simulink model "Main"  (R2020b)
settings: Solver=FixedStepAuto  StartTime=0.0  StopTime=10  FixedStep=0.01  RelTol=1e-3
libraries: TcSimInterface x1
(part 1 of 2)
settings Model: Creator=kaebi  LastModifiedBy=kaebi
settings OptimizationCC: DefaultParameterBehavior=Inlined  LocalBlockOutputs=off
settings RTWCC: Description=TwinCAT GRT Target  SystemTargetFile=TwinCatGrt.tlc  GenCodeOnly=on  TemplateMakefile=tcgrt_msbuild.tmf  TargetLang=C++
settings STFCustomTargetCC: TargetLangStandard=C++03 (ISO)  ConcurrentExecutionCompliant=off  CombineOutputUpdateFcns=on  CodeInterfacePackaging=Reusable function  GRTInterface=off  GenerateAllocFcn=on  SystemTargetFile=TwinCatGrt.tlc
settings GRTTargetCC: TargetLangStandard=C++03 (ISO)  ParMdlRefBuildCompliant=off  CompOptLevelCompliant=off  ConcurrentExecutionCompliant=off  MatFileLogging=off  CodeInterfacePackaging=Reusable function  GenerateAllocFcn=on  UseToolchainInfoCompliant=off  ExtModeMexFile=TcExtModeClient

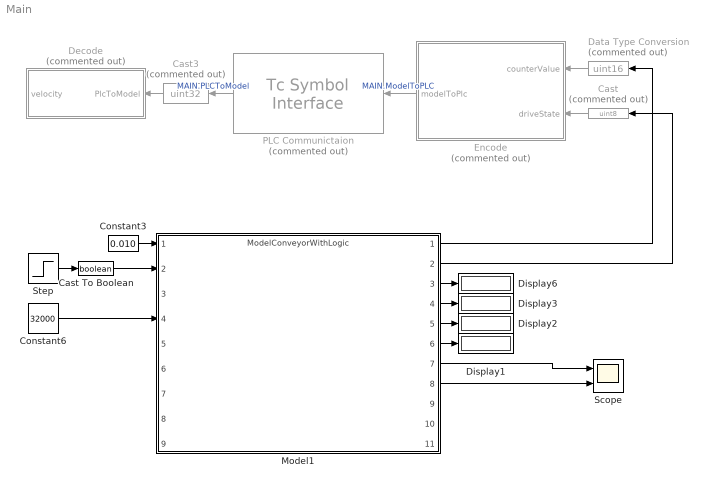
== system Main ==
  Cast : DataTypeConversion  Commented=on  OutDataTypeStr=uint8
  Cast To Boolean : DataTypeConversion  OutDataTypeStr=boolean
  Cast3 : DataTypeConversion  Commented=on  OutDataTypeStr=uint32
  Constant3 : Constant  Value=0.010
  Constant6 : Constant  Value=32000  OutDataTypeStr=int16
  Data Type Conversion : DataTypeConversion  Commented=on  OutDataTypeStr=uint16  SaturateOnIntegerOverflow=on
  Decode : MATLAB Function  Commented=on  TreatAsAtomicUnit=on
  Display{1..3,6} (4 alike) : Display
  Encode : MATLAB Function  Commented=on  TreatAsAtomicUnit=on
  Model1 : ModelReference  ModelNameDialog=ModelConveyorWithLogic.slx  SimulationMode=Normal  ModelReferenceVersion=1.29
  PLC Communictaion : TcSimInterface/Tc Symbol Interface  Commented=on  ChangeRowColOrder=on  TraceMode=3  DirectFeedThrough=0  SignalLabels=3  PortLabels=2  ExpandBusObjDepth=on  RuntimeConfig=|  SymbolInterfaceInfo=|  SyncClockMode=1
      RuntimeConfig=|
      | <?xml version="1.0" encoding="UTF-8" standalone="no"?>
      | <TcRuntimAdapterProject>
      | 	<DataTypes>
      | 		<DataType>
      | 			<Name GUID="{9165C8A1-78D1-4B81-89D0-BA48F61AF93B}" Namespace="TcDataExchange">ITcStreamSynchronizer</Name>
      | 			<Comment TxtId=""><![CDATA[Provides time synchronisation between data sources and data sinks in different time contexts. A time context might be a real time TwinCAT system the simulation time of a simulation tool or the basic time stamp of logged data in a database.]]></Comment>
      | 			<BitSize X64="64">32</BitSize>
      | 			<BaseType GUID="{00000001-0000-0000-E000-000000000064}">ITcUnknown</BaseType>
      | 			<Method>
      | 				<Name>RegisterTimeContext</Name>
      | 				<Comment><![CDATA[Registers a time context for synchronization. Registration has to be completet for all time contexts before starting the communication. ]]></Comment>
      | 				<ReturnType GUID="{18071995-0000-0000-0000-000000000019}">HRESULT</ReturnType>
      | 				<ReturnBitSize>32</ReturnBitSize>
      | 				<Parameter>
      | 					<Name>pSyncId</Name>
      | 					<Comment><![CDATA[Unique identifier of the time context. This might be e.g. the AmsNetId of a TwinCAT system or a ULINT representation of a logged dataset.]]></Comment>
      | 					<Type GUID="{18071995-0000-0000-0000-000000000021}" PointerTo="1">GUID</Type>
      | 					<BitSize X64="64">32</BitSize>
      | 				</Parameter>
      | 				<Parameter>
      | 					<Name>timeStamp</Name>
      | 					<Comment><![CDATA[Timestamp of the first received sample]]></Comment>
      | 					<Type GUID="{18071995-0000-0000-0000-00000000000C}">LINT</Type>
      | 					<BitSize>64</BitSize>
      | 				</Parameter>
      | 			</Method>
      | 			<Method>
      | 				<Name>TransformTime</Name>
      | 				<ReturnType GUID="{18071995-0000-0000-0000-000000000019}">HRESULT</ReturnType>
      | 				<ReturnBitSize>32</ReturnBitSize>
      | 				<Parameter>
      | 					<Name>pSourceSyncId</Name>
      | 					<Comment><![CDATA[Unique identifier of the source time context.]]></Comment>
      | 					<Type GUID="{18071995-0000-0000-0000-000000000021}" PointerTo="1">GUID</Type>
      | 					<BitSize X64="64">32</BitSize>
      | 				</Parameter>
      | 				<Parameter>
      | 					<Name>pSinkSyncId</Name>
      | 					<Comment><![CDATA[Unique identifier of the sink time context.]]></Comment>
      | 					<Type GUID="{18071995-0000-0000-0000-000000000021}" PointerTo="1">GUID</Type>
      | 					<BitSize X64="64">32</BitSize>
      | 				</Parameter>
      | 				<Parameter>
      | 					<Name>timeStamp</Name>
      | 					<Comment><![CDATA[Expects the sink timestamp and returns the appropriate source timestamp.
      | If the specified sink sync ID is unknown, the sink timestamp is register as its start time.]]></Comment>
      | 					<Type GUID="{18071995-0000-0000-0000-00000000000C}" ReferenceTo="true">LINT</Type>
      | 					<BitSize X64="64">32</BitSize>
      | 				</Parameter>
      | 			</Method>
      | 			<Hides>
      | 				<Hide GUID="{92EEAEA2-3DA4-48E7-A741-8C78A0326B08}"/>
      | 				<Hide GUID="{4F229E80-CBB0-4042-863E-770932FFF733}"/>
      | 				<Hide GUID="{BDB7FF6F-6144-4421-92B4-18BEEF6031E5}"/>
      | 				<Hide GUID="{5983EBFA-553B-4573-BA8B-8294D34A7664}"/>
      | 				<Hide GUID="{8DB2BF24-3BB5-46A0-91E8-A1C18BBD84A4}"/>
      | 				<Hide GUID="{865BE9CA-A112-4D69-9BA4-637F3C45508E}"/>
      | 				<Hide GUID="{5732FA65-993E-4C75-A424-0F55737580DD}"/>
      | 				<Hide GUID="{E7473B34-EFDE-47D8-AEF4-4BDF09E5E870}"/>
      | 				<Hide GUID="{BA2BDE8E-989A-4914-98EA-E301FA5E0803}"/>
      | 				<Hide GUID="{59CDFCE5-FBBF-47C8-A338-68414C56327E}"/>
      | 				<Hide GUID="{0C52276D-0720-4AEF-8258-67851E35C9C8}"/>
      | 				<Hide GUID="{4A5DD8C7-96C5-4D47-A240-8E493B9287A7}"/>
      | 			</Hides>
      | 		</DataType>
      | 		<DataType>
      | 			<Name GUID="{EA8975F7-A358-4090-8A68-57EC94D47710}" Namespace="TcDataExchange">SampleCopyInfo</Name>
      | 			<BitSize X64="192">160</BitSize>
      | 			<SubItem>
      | 				<Name>PData</Name>
      | 				<Type GUID="{18071995-0000-0000-0000-000000000001}" PointerTo="1">BYTE</Type>
      | 				<BitSize X64="64">32</BitSize>
      | 				<BitOffs>0</BitOffs>
      | 			</SubItem>
      | 			<SubItem>
      | 				<Name>CbData</Name>
      | 				<Type GUID="{18071995-0000-0000-0000-000000000008}">UDINT</Type>
      | 				<BitSize>32</BitSize>
      | 				<BitOffs X64="64">32</BitOffs>
      | 			</SubItem>
      | 			<SubItem>
      | 				<Name>ErrorCode</Name>
      | 				<Type GUID="{18071995-0000-0000-0000-000000000009}">DINT</Type>
      | 				<BitSize>32</BitSize>
      | 				<BitOffs X64="96">64</BitOffs>
      | 			</SubItem>
      | 			<SubItem>
      | 				<Name>Timestamp</Name>
      | 				<Type GUID="{18071995-0000-0000-0000-00000000000C}">LINT</Type>
      | 				<BitSize>64</BitSize>
      | 				<BitOffs X64="128">96</BitOffs>
      | 			</SubItem>
      | 			<Hides>
      | 				<Hide GUID="{97351DCE-1E32-4BD2-BF27-53E71AD5C45D}"/>
      | 				<Hide GUID="{ED3F58EE-1A95-40F4-94DA-D825E6682038}"/>
      | 				<Hide GUID="{82197966-3CEC-4E84-8982-F64641125942}"/>
      | 			</Hides>
      | 		</DataType>
      | 		<DataType>
      | 			<Name GUID="{CD026BE9-DD1E-4238-B09F-CDE426934EFB}" Namespace="TcDataExchange">ITcStreamSyncDataSink</Name>
      | 			<BitSize X64="64">32</BitSize>
      | 			<BaseType GUID="{00000001-0000-0000-E000-000000000064}">ITcUnknown</BaseType>
      | 			<Method>
      | 				<Name>WriteSamples</Name>
      | 				<ReturnType GUID="{18071995-0000-0000-0000-000000000019}">HRESULT</ReturnType>
      | 				<ReturnBitSize>32</ReturnBitSize>
      | 				<Parameter>
      | 					<Name>writerOid</Name>
      | 					<Type GUID="{18071995-0000-0000-0000-00000000000F}">OTCID</Type>
      | 					<BitSize>32</BitSize>
      | 				</Parameter>
      | 				<Parameter>
      | 					<Name>pSyncId</Name>
      | 					<Comment><![CDATA[Unique identifier of the time context. This might be e.g. the AmsNetId of a TwinCAT system or a ULINT representation of a logged dataset.]]></Comment>
      | 					<Type GUID="{18071995-0000-0000-0000-000000000021}" PointerTo="1" RpcDirection="in">GUID</Type>
      | 					<BitSize X64="64">32</BitSize>
      | 				</Parameter>
      | 				<Parameter>
      | 					<Name>sampleSize</Name>
      | 					<Type GUID="{18071995-0000-0000-0000-000000000008}" RpcDirection="in">UDINT</Type>
      | 					<BitSize>32</BitSize>
      | 				</Parameter>
      | 				<Parameter>
      | 					<Name>sampleCount</Name>
      | 					<Type GUID="{18071995-0000-0000-0000-000000000008}" RpcDirection="in">UDINT</Type>
      | 					<BitSize>32</BitSize>
      | 				</Parameter>
      | 				<Parameter>
      | 					<Name>pSamples</Name>
      | 					<Type GUID="{18071995-0000-0000-0000-000000000001}" PointerTo="1" RpcDirection="in">BYTE</Type>
      | 					<BitSize X64="64">32</BitSize>
      | 				</Parameter>
      | 				<Parameter>
      | 					<Name>pErrorCodes</Name>
      | 					<Type GUID="{18071995-0000-0000-0000-000000000009}" PointerTo="1" RpcDirection="in" RpcLengthIs="sampleCount" Optional="0">DINT</Type>
      | 					<BitSize X64="64">32</BitSize>
      | 				</Parameter>
      | 				<Parameter>
      | 					<Name>pTimeStamps</Name>
      | 					<Type GUID="{18071995-0000-0000-0000-00000000000C}" PointerTo="1" RpcDirection="in" Optional="0">LINT</Type>
      | 					<BitSize X64="64">32</BitSize>
      | 				</Parameter>
      | 				<Parameter>
      | 					<Name>sampleStride</Name>
      | 					<Type GUID="{18071995-0000-0000-0000-000000000006}" Optional="-1">INT</Type>
      | 					<BitSize>16</BitSize>
      | 				</Parameter>
      | 				<Parameter>
      | 					<Name>errorCodeStride</Name>
      | 					<Type GUID="{18071995-0000-0000-0000-000000000006}" Optional="-1">INT</Type>
      | 					<BitSize>16</BitSize>
      | 				</Parameter>
      | 				<Parameter>
      | 					<Name>timeStampStride</Name>
      | 					<Type GUID="{18071995-0000-0000-0000-000000000006}" Optional="-1">INT</Type>
      | 					<BitSize>16</BitSize>
      | 				</Parameter>
      | 			</Method>
      | 			<Method>
      | 				<Name>WriteSamples</Name>
      | 				<ReturnType GUID="{18071995-0000-0000-0000-000000000019}">HRESULT</ReturnType>
      | 				<ReturnBitSize>32</ReturnBitSize>
      | 				<Parameter>
      | 					<Name>pSyncId</Name>
      | 					<Comment><![CDATA[Unique identifier of the time context. This might be e.g. the AmsNetId of a TwinCAT system or a ULINT representation of a logged dataset.]]></Comment>
      | 					<Type GUID="{18071995-0000-0000-0000-000000000021}" PointerTo="1" RpcDirection="in">GUID</Type>
      | 					<BitSize X64="64">32</BitSize>
      | 				</Parameter>
      | 				<Parameter>
      | 					<Name>sampleCount</Name>
      | 					<Type GUID="{18071995-0000-0000-0000-000000000008}" RpcDirection="in">UDINT</Type>
      | 					<BitSize>32</BitSize>
      | 				</Parameter>
      | 				<Parameter>
      | 					<Name>pSampleCopyInfo</Name>
      | 					<Type GUID="{EA8975F7-A358-4090-8A68-57EC94D47710}" Namespace="TcDataExchange" PointerTo="1" RpcDirection="in">SampleCopyInfo</Type>
      | 					<BitSize X64="64">32</BitSize>
      | 				</Parameter>
      | 			</Method>
      | 			<Method>
      | 				<Name>GetSynchronizer</Name>
      | 				<ReturnType GUID="{18071995-0000-0000-0000-000000000019}">HRESULT</ReturnType>
      | 				<ReturnBitSize>32</ReturnBitSize>
      | 				<Parameter>
      | 					<Name>ppSynchronizer</Name>
      | 					<Type GUID="{9165C8A1-78D1-4B81-89D0-BA48F61AF93B}" Namespace="TcDataExchange" PointerTo="1">ITcStreamSynchronizer</Type>
      | 					<BitSize X64="64">32</BitSize>
      | 				</Parameter>
      | 			</Method>
      | 			<Hides>
      | 				<Hide GUID="{81DCA55F-6320-4831-9AAA-FA43AB137432}"/>
      | 				<Hide GUID="{7F649ADE-4559-4067-8B4B-52A9AFF9D566}"/>
      | 				<Hide GUID="{1ACFD07C-85DE-4584-B8DF-DCE4B2186A56}"/>
      | 				<Hide GUID="{001A190B-B452-4F64-99FE-587E5CB0E1C9}"/>
      | 				<Hide GUID="{D321BA65-82B7-4E6F-9E21-63A2CF6BE6E4}"/>
      | 				<Hide GUID="{59469964-9185-47B0-8E1F-A41A5243C9A7}"/>
      | 				<Hide GUID="{50E978C6-91D0-425B-941B-FF6E10C52E19}"/>
      | 				<Hide GUID="{2B2E9620-3973-41C2-927F-D2660E0236D6}"/>
      | 				<Hide GUID="{4C925035-5840-4BD6-BA08-B62ECBE72975}"/>
      | 				<Hide GUID="{C77882D3-FF3C-4E62-96AB-AB67CC7FA3B0}"/>
      | 				<Hide GUID="{C77882D3-FF3C-4E62-96AB-AB67CC7FA3B0}"/>
      | 				<Hide GUID="{C77882D3-FF3C-4E62-96AB-AB67CC7FA3B0}"/>
      | 				<Hide GUID="{7619FBA7-E9CC-47D7-AEE2-2BAE64602CA0}"/>
      | 				<Hide GUID="{CACC088B-451D-4181-939C-F28316D26AF6}"/>
      | 				<Hide GUID="{1701C290-46E1-4294-AA28-C9384682A3D1}"/>
      | 				<Hide GUID="{D4FE94A8-2959-45FC-B97D-A36FE755F217}"/>
      | 				<Hide GUID="{62A55225-FD8F-4450-A003-5E82394FD0D1}"/>
      | 				<Hide GUID="{7DA0071B-E1EB-4FCF-B5BE-180B5FA4841C}"/>
      | 				<Hide GUID="{D2B3A2BF-4D63-4F61-853F-3333868D1C42}"/>
      | 				<Hide GUID="{C8B9397B-AE09-4B06-8883-D01BD9BBDEFB}"/>
      | 				<Hide GUID="{276A390F-8541-45D2-8A94-8E3B6B609E81}"/>
      | 				<Hide GUID="{F4C49966-BC54-424E-A3C6-69D9FBDDE2BC}"/>
      | 			</Hides>
      | 		</DataType>
      | 		<DataType>
      | 			<Name GUID="{877CB26F-4EC1-469B-9F87-706DDBDA821F}" Namespace="TcDataExchange">ITcStreamSyncDataSource</Name>
      | 			<BitSize X64="64">32</BitSize>
      | 			<BaseType GUID="{00000001-0000-0000-E000-000000000064}">ITcUnknown</BaseType>
      | 			<Method>
      | 				<Name>ReadSamples</Name>
      | 				<ReturnType GUID="{18071995-0000-0000-0000-000000000019}">HRESULT</ReturnType>
      | 				<ReturnBitSize>32</ReturnBitSize>
      | 				<Parameter>
      | 					<Name>readerOid</Name>
      | 					<Type GUID="{18071995-0000-0000-0000-00000000000F}">OTCID</Type>
      | 					<BitSize>32</BitSize>
      | 				</Parameter>
      | 				<Parameter>
      | 					<Name>pSyncId</Name>
      | 					<Comment><![CDATA[Unique identifier of the time context. This might be e.g. the AmsNetId of a TwinCAT system or a ULINT representation of a logged dataset.]]></Comment>
      | 					<Type GUID="{18071995-0000-0000-0000-000000000021}" PointerTo="1" RpcDirection="in">GUID</Type>
      | 					<BitSize X64="64">32</BitSize>
      | 				</Parameter>
      | 				<Parameter>
      | 					<Name>sampleSize</Name>
      | 					<Type GUID="{18071995-0000-0000-0000-000000000008}" RpcDirection="in">UDINT</Type>
      | 					<BitSize>32</BitSize>
      | 				</Parameter>
      | 				<Parameter>
      | 					<Name>sampleCount</Name>
      | 					<Type GUID="{18071995-0000-0000-0000-000000000008}" ReferenceTo="true" RpcDirection="in">UDINT</Type>
      | 					<BitSize X64="64">32</BitSize>
      | 				</Parameter>
      | 				<Parameter>
      | 					<Name>pSamples</Name>
      | 					<Type GUID="{18071995-0000-0000-0000-000000000001}" PointerTo="1" RpcDirection="out">BYTE</Type>
      | 					<BitSize X64="64">32</BitSize>
      | 				</Parameter>
      | 				<Parameter>
      | 					<Name>pErrorCodes</Name>
      | 					<Type GUID="{18071995-0000-0000-0000-000000000009}" PointerTo="1" RpcDirection="out" RpcLengthIs="sampleCount" Optional="0">DINT</Type>
      | 					<BitSize X64="64">32</BitSize>
      | 				</Parameter>
      | 				<Parameter>
      | 					<Name>pTimeStamps</Name>
      | 					<Type GUID="{18071995-0000-0000-0000-00000000000C}" PointerTo="1" RpcDirection="out" RpcLengthIs="sampleCount" Optional="0">LINT</Type>
      | 					<BitSize X64="64">32</BitSize>
      | 				</Parameter>
      | 				<Parameter>
      | 					<Name>timeStamp</Name>
      | 					<Type GUID="{18071995-0000-0000-0000-00000000000C}" Optional="0">LINT</Type>
      | 					<BitSize>64</BitSize>
      | 				</Parameter>
      | 				<Parameter>
      | 					<Name>nextTimeStamp</Name>
      | 					<Type GUID="{18071995-0000-0000-0000-00000000000C}" Optional="0">LINT</Type>
      | 					<BitSize>64</BitSize>
      | 				</Parameter>
      | 			</Method>
      | 			<Method>
      | 				<Name>ReadSamples</Name>
      | 				<ReturnType GUID="{18071995-0000-0000-0000-000000000019}">HRESULT</ReturnType>
      | 				<ReturnBitSize>32</ReturnBitSize>
      | 				<Parameter>
      | 					<Name>readerOid</Name>
      | 					<Type GUID="{18071995-0000-0000-0000-00000000000F}">OTCID</Type>
      | 					<BitSize>32</BitSize>
      | 				</Parameter>
      | 				<Parameter>
      | 					<Name>pSyncId</Name>
      | 					<Comment><![CDATA[Unique identifier of the time context. This might be e.g. the AmsNetId of a TwinCAT system or a ULINT representation of a logged dataset.]]></Comment>
      | 					<Type GUID="{18071995-0000-0000-0000-000000000021}" PointerTo="1" RpcDirection="in">GUID</Type>
      | 					<BitSize X64="64">32</BitSize>
      | 				</Parameter>
      | 				<Parameter>
      | 					<Name>sampleCount</Name>
      | 					<Type GUID="{18071995-0000-0000-0000-000000000008}" ReferenceTo="true" RpcDirection="in">UDINT</Type>
      | 					<BitSize X64="64">32</BitSize>
      | 				</Parameter>
      | 				<Parameter>
      | 					<Name>pSampleCopyInfo</Name>
      | 					<Type GUID="{EA8975F7-A358-4090-8A68-57EC94D47710}" Namespace="TcDataExchange" PointerTo="1" RpcLengthIs="sampleCount">SampleCopyInfo</Type>
      | 					<BitSize X64="64">32</BitSize>
      | 				</Parameter>
      | 				<Parameter>
      | 					<Name>timeStamp</Name>
      | 					<Type GUID="{18071995-0000-0000-0000-00000000000C}" Optional="0">LINT</Type>
      | 					<BitSize>64</BitSize>
      | 				</Parameter>
      | 				<Parameter>
      | 					<Name>nextTimeStamp</Name>
      | 					<Type GUID="{18071995-0000-0000-0000-00000000000C}" Optional="0">LINT</Type>
      | 					<BitSize>64</BitSize>
      | 				</Parameter>
      | 			</Method>
      | 			<Method>
      | 				<Name>ReadSample</Name>
      | 				<ReturnType GUID="{18071995-0000-0000-0000-000000000019}">HRESULT</ReturnType>
      | 				<ReturnBitSize>32</ReturnBitSize>
      | 				<Parameter>
      | 					<Name>readerOid</Name>
      | 					<Type GUID="{18071995-0000-0000-0000-00000000000F}">OTCID</Type>
      | 					<BitSize>32</BitSize>
      | 				</Parameter>
      | 				<Parameter>
      | 					<Name>pSyncId</Name>
      | 					<Comment><![CDATA[Unique identifier of the time context. This might be e.g. the AmsNetId of a TwinCAT system or a ULINT representation of a logged dataset.]]></Comment>
      | 					<Type GUID="{18071995-0000-0000-0000-000000000021}" PointerTo="1" RpcDirection="in">GUID</Type>
      | 					<BitSize X64="64">32</BitSize>
      | 				</Parameter>
      | 				<Parameter>
      | 					<Name>sampleSize</Name>
      | 					<Type GUID="{18071995-0000-0000-0000-000000000008}" RpcDirection="in">UDINT</Type>
      | 					<BitSize>32</BitSize>
      | 				</Parameter>
      | 				<Parameter>
      | 					<Name>timeStamp</Name>
      | 					<Type GUID="{18071995-0000-0000-0000-00000000000C}" RpcDirection="in">LINT</Type>
      | 					<BitSize>64</BitSize>
      | 				</Parameter>
      | 				<Parameter>
      | 					<Name>pSample</Name>
      | 					<Type GUID="{18071995-0000-0000-0000-000000000001}" PointerTo="1" RpcDirection="out">BYTE</Type>
      | 					<BitSize X64="64">32</BitSize>
      | 				</Parameter>
      | 				<Parameter>
      | 					<Name>nextTimeStamp</Name>
      | 					<Type GUID="{18071995-0000-0000-0000-00000000000C}" Optional="0">LINT</Type>
      | 					<BitSize>64</BitSize>
      | 				</Parameter>
      | 				<Parameter>
      | 					<Name>timeoutMs</Name>
      | 					<Type GUID="{18071995-0000-0000-0000-000000000006}" Optional="0">INT</Type>
      | 					<BitSize>16</BitSize>
      | 				</Parameter>
      | 			</Method>
      | 			<Method>
      | 				<Name>ReportTransferState</Name>
      | 				<ReturnType GUID="{18071995-0000-0000-0000-000000000019}">HRESULT</ReturnType>
      | 				<ReturnBitSize>32</ReturnBitSize>
      | 				<Parameter>
      | 					<Name>sampleCount</Name>
      | 					<Type GUID="{18071995-0000-0000-0000-000000000008}" RpcDirection="in">UDINT</Type>
      | 					<BitSize>32</BitSize>
      | 				</Parameter>
      | 				<Parameter>
      | 					<Name>pTimeStamps</Name>
      | 					<Type GUID="{18071995-0000-0000-0000-00000000000B}" PointerTo="1" RpcDirection="in" RpcLengthIs="sampleCount">ULINT</Type>
      | 					<BitSize X64="64">32</BitSize>
      | 				</Parameter>
      | 				<Parameter>
      | 					<Name>pErrorCodes</Name>
      | 					<Type GUID="{18071995-0000-0000-0000-000000000009}" PointerTo="1" RpcDirection="in" RpcLengthIs="sampleCount">DINT</Type>
      | 					<BitSize X64="64">32</BitSize>
      | 				</Parameter>
      | 			</Method>
      | 			<Hides>
      | 				<Hide GUID="{82F08223-5E24-40E3-9A21-D5759118CBB7}"/>
      | 				<Hide GUID="{BC021C3C-19AB-41D1-A0EC-9FBFBB8814F1}"/>
      | 				<Hide GUID="{50FC6FF1-2968-4C30-A0C6-937238137C4E}"/>
      | 				<Hide GUID="{728E78FA-EADA-4107-BAE9-D37F8F7B9F91}"/>
      | 				<Hide GUID="{C24D9FA7-A6FF-412B-8385-D45B3613DB25}"/>
      | 				<Hide GUID="{57723EE7-8620-4304-9DD4-46EA4C8A93FC}"/>
      | 				<Hide GUID="{F29D82E8-B39D-4DDA-9326-A3CDC9CBBA4B}"/>
      | 				<Hide GUID="{53ABEA21-7053-4CE3-9300-41FAB67AF005}"/>
      | 				<Hide GUID="{E5414156-6DAA-44BD-9EFA-B9044BBB9FAE}"/>
      | 				<Hide GUID="{160EC4BE-B114-439C-A4F5-197C13AE54BE}"/>
      | 				<Hide GUID="{D7DC26B1-9810-47CC-88D8-D4B09543C26B}"/>
      | 				<Hide GUID="{2F3D2A75-7CFD-4B59-86BD-5AB92BFF5C6C}"/>
      | 				<Hide GUID="{205321E8-A331-4955-8C9E-2D60B6EAF5D8}"/>
      | 				<Hide GUID="{2F3D2A75-7CFD-4B59-86BD-5AB92BFF5C6C}"/>
      | 				<Hide GUID="{2F3D2A75-7CFD-4B59-86BD-5AB92BFF5C6C}"/>
      | 				<Hide GUID="{BA3232D2-3C23-413B-A027-D772D0C5AA3E}"/>
      | 				<Hide GUID="{FAF64FB6-67DC-4FA2-8863-A3D939045635}"/>
      | 				<Hide GUID="{5DF157ED-EE29-443B-ACD3-F7E4A686CAC8}"/>
      | 				<Hide GUID="{E20D9512-3189-4583-A5D1-6C522392AD43}"/>
      | 				<Hide GUID="{F98C9E94-47EC-40AD-AC60-E0D0FB029194}"/>
      | 				<Hide GUID="{4ED484EC-9FA9-4567-9D83-41D6BB37A214}"/>
      | 				<Hide GUID="{48244BB5-38E0-4EC3-BEA8-67AE38BFA0E5}"/>
      | 				<Hide GUID="{D85B01E0-4969-4DCF-BE5B-BBCBD9E96328}"/>
      | 				<Hide GUID="{DF45952D-9A36-4D45-934F-003F97EE2709}"/>
      | 				<Hide GUID="{582175E1-C08A-4DA1-8055-83DB0709413E}"/>
      | 				<Hide GUID="{292D2B8D-7D29-4791-A738-0FA706E6D7C7}"/>
      | 				<Hide GUID="{9660BF40-2F53-4366-912D-5DA5488BD995}"/>
      | 				<Hide GUID="{AA37253E-123B-4A23-88B2-320766B046C5}"/>
      | 				<Hide GUID="{8A9F48A1-52FB-47FA-AF47-A72CB42C8F27}"/>
      | 				<Hide GUID="{DC5918CB-E382-4038-B2ED-00FF581EA40F}"/>
      | 				<Hide GUID="{754FA08E-4EE5-4772-B861-C4D9514E5FE2}"/>
      | 				<Hide GUID="{2C0F86D1-13AC-46DB-BFB0-A62CF0B8CEE8}"/>
      | 			</Hides>
      | 		</DataType>
      | 		<DataType>
      | 			<Name GUID="{712C4007-E066-41A9-A596-8BCB41B96165}" Namespace="TcDataExchange">ITcStreamBufferEventHandler</Name>
      | 			<BitSize X64="64">32</BitSize>
      | 			<BaseType GUID="{00000001-0000-0000-E000-000000000064}">ITcUnknown</BaseType>
      | 			<Method>
      | 				<Name>Received</Name>
      | 				<ReturnType GUID="{18071995-0000-0000-0000-000000000019}">HRESULT</ReturnType>
      | 				<ReturnBitSize>32</ReturnBitSize>
      | 				<Parameter>
      | 					<Name>sampleCount</Name>
      | 					<Type GUID="{18071995-0000-0000-0000-000000000008}">UDINT</Type>
      | 					<BitSize>32</BitSize>
      | 				</Parameter>
      | 			</Method>
      | 			<Method>
      | 				<Name>Error</Name>
      | 				<ReturnType GUID="{18071995-0000-0000-0000-000000000019}">HRESULT</ReturnType>
      | 				<ReturnBitSize>32</ReturnBitSize>
      | 				<Parameter>
      | 					<Name>errorCode</Name>
      | 					<Type GUID="{18071995-0000-0000-0000-000000000008}">UDINT</Type>
      | 					<BitSize>32</BitSize>
      | 				</Parameter>
      | 			</Method>
      | 			<Method>
      | 				<Name>Overflow</Name>
      | 				<ReturnType GUID="{18071995-0000-0000-0000-000000000019}">HRESULT</ReturnType>
      | 				<ReturnBitSize>32</ReturnBitSize>
      | 				<Parameter>
      | 					<Name>overflowSamples</Name>
      | 					<Type GUID="{18071995-0000-0000-0000-000000000008}">UDINT</Type>
      | 					<BitSize>32</BitSize>
      | 				</Parameter>
      | 			</Method>
      | 			<Method>
      | 				<Name>Underflow</Name>
      | 				<ReturnType GUID="{18071995-0000-0000-0000-000000000019}">HRESULT</ReturnType>
      | 				<ReturnBitSize>32</ReturnBitSize>
      | 				<Parameter>
      | 					<Name>underflowSamples</Name>
      | 					<Type GUID="{18071995-0000-0000-0000-000000000008}">UDINT</Type>
      | 					<BitSize>32</BitSize>
      | 				</Parameter>
      | 			</Method>
      | 			<Hides>
      | 				<Hide GUID="{9693DC0A-E08C-4790-821E-EFF4431E677A}"/>
      | 				<Hide GUID="{1684DB9C-0051-460E-A769-C48582875FD5}"/>
      | 				<Hide GUID="{29D833BF-2DFE-4626-83F0-2FE339E854B3}"/>
      | 				<Hide GUID="{A287CE5A-0DB1-44AA-A6F4-1749700A23F2}"/>
      | 			</Hides>
      | 		</DataType>
      | 		<DataType>
      | 			<Name GUID="{CC2323D2-5F91-43AC-9820-54D42A9D0317}" Namespace="TcDataExchange">ITcStreamBuffer</Name>
      | 			<BitSize X64="64">32</BitSize>
      | 			<BaseType GUID="{00000001-0000-0000-E000-000000000064}">ITcUnknown</BaseType>
      | 			<Method>
      | 				<Name>RegisterEvent</Name>
      | 				<ReturnType GUID="{18071995-0000-0000-0000-000000000019}">HRESULT</ReturnType>
      | 				<ReturnBitSize>32</ReturnBitSize>
      | 				<Parameter>
      | 					<Name>pEventHandler</Name>
      | 					<Type GUID="{712C4007-E066-41A9-A596-8BCB41B96165}" Namespace="TcDataExchange">ITcStreamBufferEventHandler</Type>
      | 					<BitSize X64="64">32</BitSize>
      | 				</Parameter>
      | 				<Parameter>
      | 					<Name>nSampleCount</Name>
      | 					<Type GUID="{18071995-0000-0000-0000-000000000008}">UDINT</Type>
      | 					<BitSize>32</BitSize>
      | 				</Parameter>
      | 			</Method>
      | 			<Method>
      | 				<Name>UnregisterEvent</Name>
      | 				<ReturnType GUID="{18071995-0000-0000-0000-000000000019}">HRESULT</ReturnType>
      | 				<ReturnBitSize>32</ReturnBitSize>
      | 				<Parameter>
      | 					<Name>pEventHandler</Name>
      | 					<Type GUID="{712C4007-E066-41A9-A596-8BCB41B96165}" Namespace="TcDataExchange">ITcStreamBufferEventHandler</Type>
      | 					<BitSize X64="64">32</BitSize>
      | 				</Parameter>
      | 			</Method>
      | 			<Method>
      | 				<Name>GetSampleSize</Name>
      | 				<ReturnType GUID="{18071995-0000-0000-0000-000000000019}">HRESULT</ReturnType>
      | 				<ReturnBitSize>32</ReturnBitSize>
      | 				<Parameter>
      | 					<Name>sampleSize</Name>
      | 					<Comment><![CDATA[Byte size per sample.]]></Comment>
      | 					<Type GUID="{18071995-0000-0000-0000-000000000008}" ReferenceTo="true">UDINT</Type>
      | 					<BitSize X64="64">32</BitSize>
      | 				</Parameter>
      | 			</Method>
      | 			<Method>
      | 				<Name>GetBufferSize</Name>
      | 				<ReturnType GUID="{18071995-0000-0000-0000-000000000019}">HRESULT</ReturnType>
      | 				<ReturnBitSize>32</ReturnBitSize>
      | 				<Parameter>
      | 					<Name>bufferSize</Name>
      | 					<Comment><![CDATA[Maximum sample count.]]></Comment>
      | 					<Type GUID="{18071995-0000-0000-0000-000000000008}" ReferenceTo="true">UDINT</Type>
      | 					<BitSize X64="64">32</BitSize>
      | 				</Parameter>
      | 			</Method>
      | 			<Method>
      | 				<Name>GetUsedBufferSize</Name>
      | 				<ReturnType GUID="{18071995-0000-0000-0000-000000000019}">HRESULT</ReturnType>
      | 				<ReturnBitSize>32</ReturnBitSize>
      | 				<Parameter>
      | 					<Name>usedBufferSize</Name>
      | 					<Comment><![CDATA[Used sample count.]]></Comment>
      | 					<Type GUID="{18071995-0000-0000-0000-000000000008}" ReferenceTo="true">UDINT</Type>
      | 					<BitSize X64="64">32</BitSize>
      | 				</Parameter>
      | 			</Method>
      | 			<Hides>
      | 				<Hide GUID="{427268C9-653E-4201-A597-515502567D45}"/>
      | 				<Hide GUID="{3DA59F85-7C73-4477-A5D6-7794A3B106D1}"/>
      | 				<Hide GUID="{890211E1-E080-40B5-8BB5-2DBA8F4FB36B}"/>
      | 				<Hide GUID="{0D2BA391-E989-4F3A-AA3B-7614A7BAB3A6}"/>
      | 				<Hide GUID="{85D7F331-0847-483B-89F9-5A2034920406}"/>
      | 				<Hide GUID="{BA72510B-F66B-4B1C-BE3A-A0B28B6CB5CF}"/>
      | 			</Hides>
      | 		</DataType>
      | 		<DataType>
      | 			<Name GUID="{04A85163-BBE2-45EF-A167-1FD20C2F2D46}" Namespace="TcDataExchange">BufferReadInterpolationMode</Name>
      | 			<BitSize>16</BitSize>
      | 			<BaseType GUID="{18071995-0000-0000-0000-000000000006}">INT</BaseType>
      | 			<EnumInfo>
      | 				<Text><![CDATA[InterpolationMode_None]]></Text>
      | 				<Enum>0</Enum>
      | 				<Comment><![CDATA[No interpolation, time stamp must match existing sample]]></Comment>
      | 			</EnumInfo>
      | 			<EnumInfo>
      | 				<Text><![CDATA[InterpolationMode_Previous]]></Text>
      | 				<Enum>1</Enum>
      | 				<Comment><![CDATA[Take previous sample point]]></Comment>
      | 			</EnumInfo>
      | 			<EnumInfo>
      | 				<Text><![CDATA[InterpolationMode_Next]]></Text>
      | 				<Enum>2</Enum>
      | 				<Comment><![CDATA[Take following sample point]]></Comment>
      | 			</EnumInfo>
      | 			<EnumInfo>
      | 				<Text><![CDATA[InterpolationMode_Nearest]]></Text>
      | 				<Enum>3</Enum>
      | 				<Comment><![CDATA[Take nearest sample point]]></Comment>
      | 			</EnumInfo>
      | 			<EnumInfo>
      | 				<Text><![CDATA[InterpolationMode_Linear]]></Text>
      | 				<Enum>4</Enum>
      | 				<Comment><![CDATA[Linear interpolation]]></Comment>
      | 			</EnumInfo>
      | 			<Default>
      | 				<EnumText>InterpolationMode_Nearest</EnumText>
      | 			</Default>
      | 			<Hides>
      | 				<Hide GUID="{D1CE9774-5ABF-42E5-8FE4-99F5DEE76F36}"/>
      | 				<Hide GUID="{430DDA91-6797-4E3C-84C6-A1786F8B6EA7}"/>
      | 				<Hide GUID="{24DF4C47-A5FC-4534-A4AA-304CE11CAE9A}"/>
      | 				<Hide GUID="{5367B9B1-3807-4AFC-B79A-823BBFC694FE}"/>
      | 				<Hide GUID="{36E48A81-1480-4106-A31F-8CC0D9BDE1C1}"/>
      | 				<Hide GUID="{DB809631-0BE7-4AE2-8A30-534C3D3B8C19}"/>
      | 				<Hide GUID="{139A7071-B2F7-4999-AD00-5D72B7A47D1B}"/>
      | 				<Hide GUID="{E828C0A6-3D7C-424C-B6C8-3B4EEF9C18AC}"/>
      | 			</Hides>
      | 		</DataType>
      | 		<DataType>
      | 			<Name GUID="{B2873DF7-0E9A-4371-8FDA-560A407550FC}" Namespace="TcDataExchange">BufferReadExtrapolationMode</Name>
      | 			<BitSize>16</BitSize>
      | 			<BaseType GUID="{18071995-0000-0000-0000-000000000006}">INT</BaseType>
      | 			<EnumInfo>
      | 				<Text><![CDATA[ExtrapolationMode_None]]></Text>
      | 				<Enum>0</Enum>
      | 				<Comment><![CDATA[Return error, if the timestamp is out of the specified range]]></Comment>
      | 			</EnumInfo>
      | 			<EnumInfo>
      | 				<Text><![CDATA[ExtrapolationMode_Constant]]></Text>
      | 				<Enum>1</Enum>
      | 				<Comment><![CDATA[Use nearest sample point, if timestamp is out of the specified range]]></Comment>
      | 			</EnumInfo>
      | 			<EnumInfo>
      | 				<Text><![CDATA[ExtrapolationMode_Linear]]></Text>
      | 				<Enum>2</Enum>
      | 				<Comment><![CDATA[Extrapolate linearly, if timestamp is out of the specified range]]></Comment>
      | 			</EnumInfo>
      | 			<Hides>
      | 				<Hide GUID="{183AB6B0-9D13-4268-9013-6BC144AF43F9}"/>
      | 				<Hide GUID="{58686C98-6145-45BB-A1CE-6DFAFC306DB4}"/>
      | 				<Hide GUID="{EE21BE7C-9D24-4A92-825B-B15B1919983F}"/>
      | 				<Hide GUID="{98B9A1F3-AFB0-4DDD-856E-5CCA2E73CE75}"/>
      | 				<Hide GUID="{34806592-F19E-4DDB-96DC-032ABE8197D4}"/>
      | 				<Hide GUID="{C9391145-9682-4F6A-BF6D-5FA0733C02F4}"/>
      | 				<Hide GUID="{583534AC-9A1B-48FF-99BF-216BF02010E2}"/>
      | 				<Hide GUID="{11A9C8C7-1BFF-45E1-8ABC-29E82EA5F980}"/>
      | 				<Hide GUID="{CA042772-0740-496A-85A1-AE2E06F7EE08}"/>
      | 				<Hide GUID="{7F398EF7-03C7-49DC-B4A8-778E9B813ED0}"/>
      | 				<Hide GUID="{3075835C-D37D-4F7C-8CFA-0A55974D5F50}"/>
      | 			</Hides>
      | 		</DataType>
      | 		<DataType>
      | 			<Name GUID="{D7B34C9A-90C5-4E79-A290-017678319005}" Namespace="TcDataExchange">ITcStreamAdsRequestHandler</Name>
      | 			<BitSize X64="64">32</BitSize>
      | 			<BaseType GUID="{00000001-0000-0000-E000-000000000064}">ITcUnknown</BaseType>
      | 			<Method>
      | 				<Name>Send</Name>
      | 				<ReturnType GUID="{18071995-0000-0000-0000-000000000019}">HRESULT</ReturnType>
      | 				<ReturnBitSize>32</ReturnBitSize>
      | 				<Parameter>
      | 					<Name>timeoutMs</Name>
      | 					<Type GUID="{18071995-0000-0000-0000-000000000006}" Optional="1000">INT</Type>
      | 					<BitSize>16</BitSize>
      | 				</Parameter>
      | 			</Method>
      | 			<Method>
      | 				<Name>GetResult</Name>
      | 				<ReturnType GUID="{18071995-0000-0000-0000-000000000019}">HRESULT</ReturnType>
      | 				<ReturnBitSize>32</ReturnBitSize>
      | 				<Parameter>
      | 					<Name>pErrorCode</Name>
      | 					<Type GUID="{18071995-0000-0000-0000-000000000009}" PointerTo="1" RpcDirection="out">DINT</Type>
      | 					<BitSize X64="64">32</BitSize>
      | 				</Parameter>
      | 				<Parameter>
      | 					<Name>wait</Name>
      | 					<Type GUID="{18071995-0000-0000-0000-000000000030}" Optional="0">BOOL</Type>
      | 					<BitSize>8</BitSize>
      | 				</Parameter>
      | 			</Method>
      | 			<Method>
      | 				<Name>Cancel</Name>
      | 				<ReturnType GUID="{18071995-0000-0000-0000-000000000019}">HRESULT</ReturnType>
      | 				<ReturnBitSize>32</ReturnBitSize>
      | 			</Method>
      | 			<Hides>
      | 				<Hide GUID="{D5D4EABE-5709-4F1D-A52D-DD780CF3BEE8}"/>
      | 				<Hide GUID="{96230612-048D-4927-9A3E-E69B743416F7}"/>
      | 				<Hide GUID="{F0F623C7-A650-457C-A27C-87DC2B08989E}"/>
      | 				<Hide GUID="{18FCA6B6-AFA6-45DD-BC02-F3037EA03FB7}"/>
      | 				<Hide GUID="{12AC5FFF-B3F6-4F3E-8EDD-8044D44F084F}"/>
      | 				<Hide GUID="{6CDF8435-1307-4137-94DE-D793A77839C3}"/>
      | 			</Hides>
      | 		</DataType>
      | 		<DataType>
      | 			<Name GUID="{18071995-0000-0000-0000-000000000041}" TcBaseType="true" HideSubItems="true" CName="AmsNetId">AMSNETID</Name>
      | 			<BitSize>48</BitSize>
      | 			<BaseType GUID="{18071995-0000-0000-0000-000000000001}">BYTE</BaseType>
      | 			<ArrayInfo>
      | 				<LBound>0</LBound>
      | 				<Elements>6</Elements>
      | 			</ArrayInfo>
      | 			<Format>
      | 				<Printf>%d.%d.%d.%d.%d.%d</Printf>
      | 				<Parameter>[0]</Parameter>
      | 				<Parameter>[1]</Parameter>
      | 				<Parameter>[2]</Parameter>
      | 				<Parameter>[3]</Parameter>
      | 				<Parameter>[4]</Parameter>
      | 				<Parameter>[5]</Parameter>
      | 			</Format>
      | 		</DataType>
      | 		<DataType>
      | 			<Name GUID="{18071995-0000-0000-0000-000000000042}" TcBaseType="true" CName="AmsAddr">AMSADDR</Name>
      | 			<BitSize>64</BitSize>
      | 			<SubItem>
      | 				<Name>netId</Name>
      | 				<Type GUID="{18071995-0000-0000-0000-000000000041}">AMSNETID</Type>
      | 				<BitSize>48</BitSize>
      | 				<BitOffs>0</BitOffs>
      | 			</SubItem>
      | 			<SubItem>
      | 				<Name>port</Name>
      | 				<Type GUID="{18071995-0000-0000-0000-000000000004}">WORD</Type>
      | 				<BitSize>16</BitSize>
      | 				<BitOffs>48</BitOffs>
      | 			</SubItem>
      | 			<Format>
      | 				<Printf>%d.%d.%d.%d.%d.%d:%d</Printf>
      | 				<Parameter>.netId[0]</Parameter>
      | 				<Parameter>.netId[1]</Parameter>
      | 				<Parameter>.netId[2]</Parameter>
      | 				<Parameter>.netId[3]</Parameter>
      | 				<Parameter>.netId[4]</Parameter>
      | 				<Parameter>.netId[5]</Parameter>
      | 				<Parameter>.port</Parameter>
      | 			</Format>
      | 			<Format Name="Iec">
      | 				<Printf>(netId:=[%d.%d.%d.%d.%d.%d], port :=%d)</Printf>
      | 				<Parameter>.netId[0]</Parameter>
      | 				<Parameter>.netId[1]</Parameter>
      | 				<Parameter>.netId[2]</Parameter>
      | 				<Parameter>.netId[3]</Parameter>
      | 				<Parameter>.netId[4]</Parameter>
      | 				<Parameter>.netId[5]</Parameter>
      | 				<Parameter>.port</Parameter>
      | 			</Format>
      | 		</DataType>
      | 		<DataType>
      | 			<Name GUID="{2919D6B4-47C4-4AE8-B706-E94C497ECB99}" Namespace="TcDataExchange">NotificationTransMode</Name>
      | 			<BitSize>16</BitSize>
      | 			<BaseType GUID="{18071995-0000-0000-0000-000000000006}">INT</BaseType>
      | 			<EnumInfo>
      | 				<Text><![CDATA[NoTrans]]></Text>
      | 				<Enum>0</Enum>
      | 			</EnumInfo>
      | 			<EnumInfo>
      | 				<Text><![CDATA[ServerCycle]]></Text>
      | 				<Enum>3</Enum>
      | 			</EnumInfo>
      | 			<EnumInfo>
      | 				<Text><![CDATA[OnChange]]></Text>
      | 				<Enum>4</Enum>
      | 			</EnumInfo>
      | 			<Hides>
      | 				<Hide GUID="{79465139-46B4-43EB-B7FF-967BF64C3367}"/>
      | 				<Hide GUID="{AE2F4BB5-B98E-4C79-AC26-086A9CF7EAC6}"/>
      | 				<Hide GUID="{ECF929B2-79C7-483F-A3DC-06B91AFD531C}"/>
      | 				<Hide GUID="{4E4B27B2-E550-42F1-92B6-1EFABDB0481B}"/>
      | 			</Hides>
      | 		</DataType>
      | 		<DataType>
      | 			<Name GUID="{B75DDCED-7BC8-45F5-8D80-27345642612D}" Namespace="TcDataExchange">NotificationState</Name>
      | 			<BitSize>16</BitSize>
      | 			<BaseType GUID="{18071995-0000-0000-0000-000000000006}">INT</BaseType>
      | 			<EnumInfo>
      | 				<Text><![CDATA[Stop]]></Text>
      | 				<Enum>0</Enum>
      | 			</EnumInfo>
      | 			<EnumInfo>
      | 				<Text><![CDATA[Starting]]></Text>
      | 				<Enum>1</Enum>
      | 			</EnumInfo>
      | 			<EnumInfo>
      | 				<Text><![CDATA[Run]]></Text>
      | 				<Enum>2</Enum>
      | 			</EnumInfo>
      | 			<EnumInfo>
      | 				<Text><![CDATA[Stopping]]></Text>
      | 				<Enum>3</Enum>
      | 			</EnumInfo>
      | 			<EnumInfo>
      | 				<Text><![CDATA[StartError]]></Text>
      | 				<Enum>4</Enum>
      | 			</EnumInfo>
      | 			<EnumInfo>
      | 				<Text><![CDATA[StopError]]></Text>
      | 				<Enum>5</Enum>
      | 			</EnumInfo>
      | 			<Hides>
      | 				<Hide GUID="{BEEA3766-C152-4B4D-80E7-6332297C102B}"/>
      | 			</Hides>
      | 		</DataType>
      | 		<DataType>
      | 			<Name GUID="{7BD2CA64-894F-4710-AF21-189254BD7339}" Namespace="TcDataExchange">ITcStreamAdsNotificationHandler</Name>
      | 			<BitSize X64="64">32</BitSize>
      | 			<BaseType GUID="{00000001-0000-0000-E000-000000000064}">ITcUnknown</BaseType>
      | 			<Method>
      | 				<Name>Start</Name>
      | 				<ReturnType GUID="{18071995-0000-0000-0000-000000000019}">HRESULT</ReturnType>
      | 				<ReturnBitSize>32</ReturnBitSize>
      | 				<Parameter>
      | 					<Name>sampleTime100ns</Name>
      | 					<Comment><![CDATA[SampleTime in 100ns. If the value is 0 or too small, the requests will be send as fast as possible.]]></Comment>
      | 					<Type GUID="{18071995-0000-0000-0000-000000000008}" Optional="0">UDINT</Type>
      | 					<BitSize>32</BitSize>
      | 				</Parameter>
      | 				<Parameter>
      | 					<Name>delayTime100ns</Name>
      | 					<Comment><![CDATA[DelayTime in 100ns.]]></Comment>
      | 					<Type GUID="{18071995-0000-0000-0000-000000000008}" Optional="10">UDINT</Type>
      | 					<BitSize>32</BitSize>
      | 				</Parameter>
      | 				<Parameter>
      | 					<Name>createTimeoutMs</Name>
      | 					<Type GUID="{18071995-0000-0000-0000-000000000006}" Optional="1000">INT</Type>
      | 					<BitSize>16</BitSize>
      | 				</Parameter>
      | 				<Parameter>
      | 					<Name>transMode</Name>
      | 					<Type GUID="{2919D6B4-47C4-4AE8-B706-E94C497ECB99}" Namespace="TcDataExchange" Optional="0">NotificationTransMode</Type>
      | 					<BitSize>16</BitSize>
      | 				</Parameter>
      | 			</Method>
      | 			<Method>
      | 				<Name>Stop</Name>
      | 				<ReturnType GUID="{18071995-0000-0000-0000-000000000019}">HRESULT</ReturnType>
      | 				<ReturnBitSize>32</ReturnBitSize>
      | 				<Parameter>
      | 					<Name>stopTimeoutMs</Name>
      | 					<Type GUID="{18071995-0000-0000-0000-000000000006}" Optional="1000">INT</Type>
      | 					<BitSize>16</BitSize>
      | 				</Parameter>
      | 			</Method>
      | 			<Method>
      | 				<Name>GetState</Name>
      | 				<ReturnType GUID="{18071995-0000-0000-0000-000000000019}">HRESULT</ReturnType>
      | 				<ReturnBitSize>32</ReturnBitSize>
      | 				<Parameter>
      | 					<Name>pState</Name>
      | 					<Type GUID="{B75DDCED-7BC8-45F5-8D80-27345642612D}" Namespace="TcDataExchange" PointerTo="1">NotificationState</Type>
      | 					<BitSize X64="64">32</BitSize>
      | 				</Parameter>
      | 				<Parameter>
      | 					<Name>pErrorCode</Name>
      | 					<Type GUID="{18071995-0000-0000-0000-000000000009}" PointerTo="1">DINT</Type>
      | 					<BitSize X64="64">32</BitSize>
      | 				</Parameter>
      | 			</Method>
      | 			<Method>
      | 				<Name>WaitFor</Name>
      | 				<ReturnType GUID="{18071995-0000-0000-0000-000000000019}">HRESULT</ReturnType>
      | 				<ReturnBitSize>32</ReturnBitSize>
      | 				<Parameter>
      | 					<Name>targetState</Name>
      | 					<Type GUID="{B75DDCED-7BC8-45F5-8D80-27345642612D}" Namespace="TcDataExchange">NotificationState</Type>
      | 					<BitSize>16</BitSize>
      | 				</Parameter>
      | 			</Method>
      | 			<Hides>
      | 				<Hide GUID="{0FD54C3A-649C-4819-BA34-40090DB2854F}"/>
      | 				<Hide GUID="{B851627D-4078-4428-873B-9E0DE756697F}"/>
      | 				<Hide GUID="{82738EA0-63AE-4386-9AC8-D5A166BE7CE6}"/>
      | 				<Hide GUID="{62C58600-337E-4913-B519-B241B47A093F}"/>
      | 				<Hide GUID="{F19E62E1-3672-44A5-AE6F-41D70903D13E}"/>
      | 				<Hide GUID="{188DFF90-A46E-4A6C-BF2A-4B79F1A4A7D7}"/>
      | 				<Hide GUID="{20D7666F-EA21-4A02-B0BF-92A2B39D0282}"/>
      | 				<Hide GUID="{B6680295-EE8B-49D4-B982-46287CB9DC7F}"/>
      | 				<Hide GUID="{640F79DB-CF38-45B7-A5A6-1F8ACF6E88C7}"/>
      | 				<Hide GUID="{ACD4E2BC-BCCF-47C3-994A-79C84DA897B4}"/>
      | 			</Hides>
      | 		</DataType>
      | 		<DataType>
      | 			<Name GUID="{44CF19E6-1A23-4E07-B15E-18C86B7D1DF6}" Namespace="TcDataExchange">ITcStreamAdsClient</Name>
      | 			<BitSize X64="64">32</BitSize>
      | 			<BaseType GUID="{00000001-0000-0000-E000-000000000064}">ITcUnknown</BaseType>
      | 			<Method>
      | 				<Name>CreateReadRequest</Name>
      | 				<ReturnType GUID="{18071995-0000-0000-0000-000000000019}">HRESULT</ReturnType>
      | 				<ReturnBitSize>32</ReturnBitSize>
      | 				<Parameter>
      | 					<Name>parentOid</Name>
      | 					<Type GUID="{18071995-0000-0000-0000-00000000000F}">OTCID</Type>
      | 					<BitSize>32</BitSize>
      | 				</Parameter>
      | 				<Parameter>
      | 					<Name>ppRequestHandler</Name>
      | 					<Type GUID="{D7B34C9A-90C5-4E79-A290-017678319005}" Namespace="TcDataExchange" PointerTo="1" RpcDirection="out">ITcStreamAdsRequestHandler</Type>
      | 					<BitSize X64="64">32</BitSize>
      | 				</Parameter>
      | 				<Parameter>
      | 					<Name>amsAddr</Name>
      | 					<Type GUID="{18071995-0000-0000-0000-000000000042}" RpcDirection="in">AMSADDR</Type>
      | 					<BitSize>64</BitSize>
      | 				</Parameter>
      | 				<Parameter>
      | 					<Name>idxGrp</Name>
      | 					<Type GUID="{18071995-0000-0000-0000-000000000008}" RpcDirection="in">UDINT</Type>
      | 					<BitSize>32</BitSize>
      | 				</Parameter>
      | 				<Parameter>
      | 					<Name>idxOffs</Name>
      | 					<Type GUID="{18071995-0000-0000-0000-000000000008}" RpcDirection="in">UDINT</Type>
      | 					<BitSize>32</BitSize>
      | 				</Parameter>
      | 				<Parameter>
      | 					<Name>byteSize</Name>
      | 					<Type GUID="{18071995-0000-0000-0000-000000000008}" RpcDirection="in">UDINT</Type>
      | 					<BitSize>32</BitSize>
      | 				</Parameter>
      | 				<Parameter>
      | 					<Name>pSink</Name>
      | 					<Type GUID="{CD026BE9-DD1E-4238-B09F-CDE426934EFB}" Namespace="TcDataExchange" RpcDirection="in">ITcStreamSyncDataSink</Type>
      | 					<BitSize X64="64">32</BitSize>
      | 				</Parameter>
      | 			</Method>
      | 			<Method>
      | 				<Name>CreateWriteRequest</Name>
      | 				<ReturnType GUID="{18071995-0000-0000-0000-000000000019}">HRESULT</ReturnType>
      | 				<ReturnBitSize>32</ReturnBitSize>
      | 				<Parameter>
      | 					<Name>parentOid</Name>
      | 					<Type GUID="{18071995-0000-0000-0000-00000000000F}">OTCID</Type>
      | 					<BitSize>32</BitSize>
      | 				</Parameter>
      | 				<Parameter>
      | 					<Name>ppRequestHandler</Name>
      | 					<Type GUID="{D7B34C9A-90C5-4E79-A290-017678319005}" Namespace="TcDataExchange" PointerTo="1" RpcDirection="out">ITcStreamAdsRequestHandler</Type>
      | 					<BitSize X64="64">32</BitSize>
      | 				</Parameter>
      | 				<Parameter>
      | 					<Name>amsAddr</Name>
      | 					<Type GUID="{18071995-0000-0000-0000-000000000042}" RpcDirection="in">AMSADDR</Type>
      | 					<BitSize>64</BitSize>
      | 				</Parameter>
      | 				<Parameter>
      | 					<Name>idxGrp</Name>
      | 					<Type GUID="{18071995-0000-0000-0000-000000000008}" RpcDirection="in">UDINT</Type>
      | 					<BitSize>32</BitSize>
      | 				</Parameter>
      | 				<Parameter>
      | 					<Name>idxOffs</Name>
      | 					<Type GUID="{18071995-0000-0000-0000-000000000008}" RpcDirection="in">UDINT</Type>
      | 					<BitSize>32</BitSize>
      | 				</Parameter>
      | 				<Parameter>
      | 					<Name>byteSize</Name>
      | 					<Type GUID="{18071995-0000-0000-0000-000000000008}" RpcDirection="in">UDINT</Type>
      | 					<BitSize>32</BitSize>
      | 				</Parameter>
      | 				<Parameter>
      | 					<Name>pSource</Name>
      | 					<Type GUID="{877CB26F-4EC1-469B-9F87-706DDBDA821F}" Namespace="TcDataExchange" RpcDirection="in">ITcStreamSyncDataSource</Type>
      | 					<BitSize X64="64">32</BitSize>
      | 				</Parameter>
      | 			</Method>
      | 			<Method>
      | 				<Name>CreateReadWriteRequest</Name>
      | 				<ReturnType GUID="{18071995-0000-0000-0000-000000000019}">HRESULT</ReturnType>
      | 				<ReturnBitSize>32</ReturnBitSize>
      | 				<Parameter>
      | 					<Name>parentOid</Name>
      | 					<Type GUID="{18071995-0000-0000-0000-00000000000F}">OTCID</Type>
      | 					<BitSize>32</BitSize>
      | 				</Parameter>
      | 				<Parameter>
      | 					<Name>ppRequestHandler</Name>
      | 					<Type GUID="{D7B34C9A-90C5-4E79-A290-017678319005}" Namespace="TcDataExchange" PointerTo="1" RpcDirection="out">ITcStreamAdsRequestHandler</Type>
      | 					<BitSize X64="64">32</BitSize>
      | 				</Parameter>
      | 				<Parameter>
      | 					<Name>amsAddr</Name>
      | 					<Type GUID="{18071995-0000-0000-0000-000000000042}" RpcDirection="in">AMSADDR</Type>
      | 					<BitSize>64</BitSize>
      | 				</Parameter>
      | 				<Parameter>
      | 					<Name>idxGrp</Name>
      | 					<Type GUID="{18071995-0000-0000-0000-000000000008}" RpcDirection="in">UDINT</Type>
      | 					<BitSize>32</BitSize>
      | 				</Parameter>
      | 				<Parameter>
      | 					<Name>idxOffs</Name>
      | 					<Type GUID="{18071995-0000-0000-0000-000000000008}" RpcDirection="in">UDINT</Type>
      | 					<BitSize>32</BitSize>
      | 				</Parameter>
      | 				<Parameter>
      | 					<Name>writeSize</Name>
      | 					<Type GUID="{18071995-0000-0000-0000-000000000008}" RpcDirection="in">UDINT</Type>
      | 					<BitSize>32</BitSize>
      | 				</Parameter>
      | 				<Parameter>
      | 					<Name>pSource</Name>
      | 					<Type GUID="{877CB26F-4EC1-469B-9F87-706DDBDA821F}" Namespace="TcDataExchange" RpcDirection="in">ITcStreamSyncDataSource</Type>
      | 					<BitSize X64="64">32</BitSize>
      | 				</Parameter>
      | 				<Parameter>
      | 					<Name>readSize</Name>
      | 					<Type GUID="{18071995-0000-0000-0000-000000000008}" RpcDirection="in">UDINT</Type>
      | 					<BitSize>32</BitSize>
      | 				</Parameter>
      | 				<Parameter>
      | 					<Name>pSink</Name>
      | 					<Type GUID="{CD026BE9-DD1E-4238-B09F-CDE426934EFB}" Namespace="TcDataExchange" RpcDirection="in">ITcStreamSyncDataSink</Type>
      | 					<BitSize X64="64">32</BitSize>
      | 				</Parameter>
      | 			</Method>
      | 			<Method>
      | 				<Name>CreateNotificationHandler</Name>
      | 				<ReturnType GUID="{18071995-0000-0000-0000-000000000019}">HRESULT</ReturnType>
      | 				<ReturnBitSize>32</ReturnBitSize>
      | 				<Parameter>
      | 					<Name>parentOid</Name>
      | 					<Type GUID="{18071995-0000-0000-0000-00000000000F}">OTCID</Type>
      | 					<BitSize>32</BitSize>
      | 				</Parameter>
      | 				<Parameter>
      | 					<Name>ppNotificationHandler</Name>
      | 					<Type GUID="{7BD2CA64-894F-4710-AF21-189254BD7339}" Namespace="TcDataExchange" PointerTo="1" RpcDirection="out">ITcStreamAdsNotificationHandler</Type>
      | 					<BitSize X64="64">32</BitSize>
      | 				</Parameter>
      | 				<Parameter>
      | 					<Name>amsAddr</Name>
      | 					<Type GUID="{18071995-0000-0000-0000-000000000042}">AMSADDR</Type>
      | 					<BitSize>64</BitSize>
      | 				</Parameter>
      | 				<Parameter>
      | 					<Name>idxGrp</Name>
      | 					<Type GUID="{18071995-0000-0000-0000-000000000008}" RpcDirection="in">UDINT</Type>
      | 					<BitSize>32</BitSize>
      | 				</Parameter>
      | 				<Parameter>
      | 					<Name>idxOffs</Name>
      | 					<Type GUID="{18071995-0000-0000-0000-000000000008}" RpcDirection="in">UDINT</Type>
      | 					<BitSize>32</BitSize>
      | 				</Parameter>
      | 				<Parameter>
      | 					<Name>byteSize</Name>
      | 					<Type GUID="{18071995-0000-0000-0000-000000000008}" RpcDirection="in">UDINT</Type>
      | 					<BitSize>32</BitSize>
      | 				</Parameter>
      | 				<Parameter>
      | 					<Name>pSink</Name>
      | 					<Type GUID="{CD026BE9-DD1E-4238-B09F-CDE426934EFB}" Namespace="TcDataExchange" RpcDirection="in">ITcStreamSyncDataSink</Type>
      | 					<BitSize X64="64">32</BitSize>
      | 				</Parameter>
      | 			</Method>
      | 			<Hides>
      | 				<Hide GUID="{E5572F78-39F4-4573-890C-3DF0E2006105}"/>
      | 				<Hide GUID="{52252529-8C17-45D1-85B4-6A458C0F3E94}"/>
      | 				<Hide GUID="{F824C7E1-F0C6-44A6-B482-897B83EFF54D}"/>
      | 				<Hide GUID="{89D1DEF9-1EDB-4DC7-B44F-67745448E326}"/>
      | 				<Hide GUID="{9AF2891A-A1C3-41B4-843B-F1318836B90C}"/>
      | 				<Hide GUID="{C92F8EE8-70FC-4938-AE5D-0804054FE778}"/>
      | 				<Hide GUID="{692D2F91-2921-429B-A2FD-B23E2D06FE57}"/>
      | 				<Hide GUID="{247F4AE9-8FC4-4311-BF3B-2963D4FB048A}"/>
      | 				<Hide GUID="{FB8AA9BF-37B4-4992-B5AC-BBA0F4D43373}"/>
      | 				<Hide GUID="{7427C36F-E349-41A6-A066-CB0C042DD556}"/>
      | 				<Hide GUID="{E46C7F48-0073-45AF-850A-7F1CB9D0F1BC}"/>
      | 				<Hide GUID="{096DB961-B576-4662-AA01-00D308385BF0}"/>
      | 				<Hide GUID="{A0AD0C9E-66BD-49F7-B782-910B430A1CD8}"/>
      | 				<Hide GUID="{FA6AC3AF-43AA-44CB-BA36-5723B1AD464D}"/>
      | 				<Hide GUID="{0614F527-21B4-4192-AE03-7FDCC97AD564}"/>
      | 				<Hide GUID="{20F9385A-0313-4208-B227-DA4EACC1424F}"/>
      | 				<Hide GUID="{DBEA0444-99ED-4B99-9B51-31DB70AF46EF}"/>
      | 				<Hide GUID="{C3B2FC5E-7AD1-45D8-9723-AA6C61AD9B60}"/>
      | 				<Hide GUID="{CF97D717-7515-4E5A-BE1F-84F5A676B8F8}"/>
      | 				<Hide GUID="{B3BDED57-1312-4D96-B06F-2628ECBA6EEF}"/>
      | 				<Hide GUID="{5DE91436-84B1-4D76-B0CA-1D6620CA428C}"/>
      | 				<Hide GUID="{A0E457C6-B984-4427-829D-FA992FA6D9F8}"/>
      | 				<Hide GUID="{49669A99-FF7E-4056-9658-FDC96AB6BD99}"/>
      | 				<Hide GUID="{53867E37-5FD2-456B-BE41-4F337E21E47A}"/>
      | 				<Hide GUID="{A3973658-0AF9-4706-9520-0AAF0F575BFE}"/>
      | 				<Hide GUID="{FC062AA8-EE46-46C7-94CF-827603675385}"/>
      | 				<Hide GUID="{021F7DA4-A9B9-4EF5-80F9-A8DBC397B675}"/>
      | 				<Hide GUID="{4D5006B6-E8E6-4498-9498-ACA7E948FC8F}"/>
      | 				<Hide GUID="{984AB404-08AC-4281-AB66-6ED5B3F17DFE}"/>
      | 				<Hide GUID="{D581F6CF-93AC-4E4B-8D6F-3F0EF3492A71}"/>
      | 				<Hide GUID="{7A32D7B0-99BA-4055-815F-11160248ACD0}"/>
      | 				<Hide GUID="{9E7FC559-CAD5-43C8-B16B-2E56C1991573}"/>
      | 				<Hide GUID="{F062CF59-8FAE-4FCB-A01C-9B649900BCA5}"/>
      | 				<Hide GUID="{8728E0D9-0A46-4A30-9F10-DD1BF2EA33CE}"/>
      | 				<Hide GUID="{DFBB006E-343D-4910-A9C8-3AB2FE1535D3}"/>
      | 				<Hide GUID="{28C016BE-C467-4209-83F6-DED24711BF6D}"/>
      | 				<Hide GUID="{090DBC60-C9BC-4AB3-B82F-77F59E060169}"/>
      | 				<Hide GUID="{7C69CB05-063E-4BC5-9379-7224930A2D33}"/>
      | 				<Hide GUID="{AFAD7A5B-01FD-4391-87A6-15283DC78C95}"/>
      | 				<Hide GUID="{5E61A921-550A-4063-9429-A8A28DE5A1E3}"/>
      | 				<Hide GUID="{6BB012C3-FEAE-471E-BD95-27EDA5BB3A24}"/>
      | 				<Hide GUID="{E5B9394C-8543-4D1E-86CA-EC772D80F874}"/>
      | 				<Hide GUID="{B8FC3674-8C27-4962-8D53-5010B3276572}"/>
      | 				<Hide GUID="{7A879166-081C-4396-83F5-1ED6DDC3FE02}"/>
      | 				<Hide GUID="{906345FE-D08D-48EB-B8DC-3909739597CB}"/>
      | 			</Hides>
      | 		</DataType>
      | 	</DataTypes>
      | 	<Translations/>
      | 	<System>
      | 		<Tasks>
      | 			<Task ObjectId="33620000" CycleTime="100000" AmsPort="350" Priority="20">
      | 				<Name>TcDataExchangeModulesTask</Name>
      | 			</Task>
      | 		</Tasks>
      | 		<Modules>
      | 			<Module GUID="{AB7EF359-EC28-4A80-B6B9-1F5FEF806409}" ClassFactoryId="Beckhoff Automation|TcDataExchangeModules|1.0.1.166" Group="DataExchange|StreamUtilities">
      | 				<Name>Synchronizer</Name>
      | 				<CLSID ClassFactory="TcDataExchangeModules">{AB7EF359-EC28-4A80-B6B9-1F5FEF806409}</CLSID>
      | 				<Info/>
      | 				<Licenses>
      | 					<License>
      | 						<LicenseId>{304D006A-8299-4560-AB79-438534B50288}</LicenseId>
      | 					</License>
      | 				</Licenses>
      | 				<InitSequence>SO</InitSequence>
      | 				<Contexts>
      | 					<Context>
      | 						<Id>1</Id>
      | 					</Context>
      | 				</Contexts>
      | 				<Interfaces>
      | 					<Interface DisableCodeGeneration="true">
      | 						<Type GUID="{00000012-0000-0000-E000-000000000064}">ITComObject</Type>
      | 					</Interface>
      | 					<Interface DisableCodeGeneration="true">
      | 						<Type GUID="{03000012-0000-0000-E000-000000000064}">ITcADI</Type>
      | 					</Interface>
      | 					<Interface DisableCodeGeneration="true">
      | 						<Type GUID="{03000018-0000-0000-E000-000000000064}">ITcWatchSource</Type>
      | 					</Interface>
      | 					<Interface>
      | 						<Type GUID="{9165C8A1-78D1-4B81-89D0-BA48F61AF93B}" Namespace="TcDataExchange">ITcStreamSynchronizer</Type>
      | 					</Interface>
      | 				</Interfaces>
      | 				<Parameters>
      | 					<Parameter HideParameter="true">
      | 						<Name>TraceLevelMax</Name>
      | 						<Comment TxtId=""><![CDATA[Controls the amount of log messages.]]></Comment>
      | 						<BitSize>32</BitSize>
      | 						<BaseType GUID="{8007AE3B-86BB-40F2-B385-EF87FCC239A4}">TcTraceLevel</BaseType>
      | 						<PTCID>#x03002103</PTCID>
      | 						<ContextId>1</ContextId>
      | 					</Parameter>
      | 				</Parameters>
      | 				<InstanceName>Synchronizer_Instance1</InstanceName>
      | 				<OTCID>#x01010010</OTCID>
      | 				<ParameterValues>
      | 					<Value>
      | 						<Name>TraceLevelMax</Name>
      | 						<EnumText>tlAlways</EnumText>
      | 					</Value>
      | 				</ParameterValues>
      | 			</Module>
      | 			<Module GUID="{7F2917A9-6092-40A6-BB22-5428D680BA27}" ClassFactoryId="Beckhoff Automation|TcDataExchangeModules|1.0.1.166" Group="DataExchange|StreamUtilities">
      | 				<Name>SyncBuffer</Name>
      | 				<CLSID ClassFactory="TcDataExchangeModules">{7F2917A9-6092-40A6-BB22-5428D680BA27}</CLSID>
      | 				<Info/>
      | 				<Licenses>
      | 					<License>
      | 						<LicenseId>{304D006A-8299-4560-AB79-438534B50288}</LicenseId>
      | 					</License>
      | 				</Licenses>
      | 				<InitSequence>SO</InitSequence>
      | 				<Contexts>
      | 					<Context>
      | 						<Id>1</Id>
      | 					</Context>
      | 				</Contexts>
      | 				<Interfaces>
      | 					<Interface DisableCodeGeneration="true">
      | 						<Type GUID="{00000012-0000-0000-E000-000000000064}">ITComObject</Type>
      | 					</Interface>
      | 					<Interface DisableCodeGeneration="true">
      | 						<Type GUID="{03000012-0000-0000-E000-000000000064}">ITcADI</Type>
      | 					</Interface>
      | 					<Interface DisableCodeGeneration="true">
      | 						<Type GUID="{03000018-0000-0000-E000-000000000064}">ITcWatchSource</Type>
      | 					</Interface>
      | 					<Interface>
      | 						<Type GUID="{CD026BE9-DD1E-4238-B09F-CDE426934EFB}" Namespace="TcDataExchange">ITcStreamSyncDataSink</Type>
      | 					</Interface>
      | 					<Interface>
      | 						<Type GUID="{877CB26F-4EC1-469B-9F87-706DDBDA821F}" Namespace="TcDataExchange">ITcStreamSyncDataSource</Type>
      | 					</Interface>
      | 					<Interface>
      | 						<Type GUID="{CC2323D2-5F91-43AC-9820-54D42A9D0317}" Namespace="TcDataExchange">ITcStreamBuffer</Type>
      | 					</Interface>
      | 				</Interfaces>
      | 				<Parameters>
      | 					<Parameter>
      | 						<Name>InterpolationMode</Name>
      | 						<BitSize>16</BitSize>
      | 						<BaseType GUID="{04A85163-BBE2-45EF-A167-1FD20C2F2D46}" Namespace="TcDataExchange">BufferReadInterpolationMode</BaseType>
      | 						<PTCID>#x00000004</PTCID>
      | 						<ContextId>1</ContextId>
      | 					</Parameter>
      | 					<Parameter>
      | 						<Name>ContinuationMode</Name>
      | 						<BitSize>16</BitSize>
      | 						<BaseType GUID="{B2873DF7-0E9A-4371-8FDA-560A407550FC}" Namespace="TcDataExchange">BufferReadExtrapolationMode</BaseType>
      | 						<PTCID>#x00000005</PTCID>
      | 						<ContextId>1</ContextId>
      | 					</Parameter>
      | 					<Parameter>
      | 						<Name>SampleSize</Name>
      | 						<BitSize>32</BitSize>
      | 						<BaseType GUID="{18071995-0000-0000-0000-000000000008}">UDINT</BaseType>
      | 						<PTCID>#x00000006</PTCID>
      | 						<ContextId>1</ContextId>
      | 					</Parameter>
      | 					<Parameter>
      | 						<Name>Capacity</Name>
      | 						<BitSize>32</BitSize>
      | 						<BaseType GUID="{18071995-0000-0000-0000-000000000008}">UDINT</BaseType>
      | 						<PTCID>#x00000007</PTCID>
      | 						<ContextId>1</ContextId>
      | 					</Parameter>
      | 					<Parameter HideParameter="true">
      | 						<Name>TraceLevelMax</Name>
      | 						<Comment TxtId=""><![CDATA[Controls the amount of log messages.]]></Comment>
      | 						<BitSize>32</BitSize>
      | 						<BaseType GUID="{8007AE3B-86BB-40F2-B385-EF87FCC239A4}">TcTraceLevel</BaseType>
      | 						<PTCID>#x03002103</PTCID>
      | 						<ContextId>1</ContextId>
      | 					</Parameter>
      | 				</Parameters>
      | 				<InterfacePointers>
      | 					<InterfacePointer>
      | 						<PTCID>#x00000001</PTCID>
      | 						<Name>Synchronizer</Name>
      | 						<Type GUID="{9165C8A1-78D1-4B81-89D0-BA48F61AF93B}" Namespace="TcDataExchange">ITcStreamSynchronizer</Type>
      | 						<ContextId>1</ContextId>
      | 					</InterfacePointer>
      | 				</InterfacePointers>
      | 				<InstanceName>SyncBuffer_Instance1</InstanceName>
      | 				<OTCID>#x01010020</OTCID>
      | 				<ParameterValues>
      | 					<Value>
      | 						<Name>InterpolationMode</Name>
      | 						<EnumText>InterpolationMode_Nearest</EnumText>
      | 					</Value>
      | 					<Value>
      | 						<Name>ContinuationMode</Name>
      | 						<EnumText>ExtrapolationMode_None</EnumText>
      | 					</Value>
      | 					<Value>
      | 						<Name>SampleSize</Name>
      | 						<Value>4</Value>
      | 					</Value>
      | 					<Value>
      | 						<Name>Capacity</Name>
      | 						<Value>50</Value>
      | 					</Value>
      | 					<Value>
      | 						<Name>TraceLevelMax</Name>
      | 						<EnumText>tlAlways</EnumText>
      | 					</Value>
      | 				</ParameterValues>
      | 				<InterfacePointerValues>
      | 					<Value>
      | 						<Name>Synchronizer</Name>
      | 						<OTCID>#x01010010</OTCID>
      | 					</Value>
      | 				</InterfacePointerValues>
      | 			</Module>
      | 			<Module GUID="{976B3EC0-C035-4B78-B648-B8952590F899}" ClassFactoryId="Beckhoff Automation|TcDataExchangeModules|1.0.1.166" Group="DataExchange|StreamSinkSource">
      | 				<Name>FromDataArea</Name>
      | 				<CLSID ClassFactory="TcDataExchangeModules">{976B3EC0-C035-4B78-B648-B8952590F899}</CLSID>
      | 				<Info/>
      | 				<Licenses>
      | 					<License>
      | 						<LicenseId>{304D006A-8299-4560-AB79-438534B50288}</LicenseId>
      | 					</License>
      | 				</Licenses>
      | 				<InitSequence>SO</InitSequence>
      | 				<Contexts>
      | 					<Context>
      | 						<Id>1</Id>
      | 					</Context>
      | 				</Contexts>
      | 				<Interfaces>
      | 					<Interface DisableCodeGeneration="true">
      | 						<Type GUID="{00000012-0000-0000-E000-000000000064}">ITComObject</Type>
      | 					</Interface>
      | 					<Interface DisableCodeGeneration="true">
      | 						<Type GUID="{03000012-0000-0000-E000-000000000064}">ITcADI</Type>
      | 					</Interface>
      | 					<Interface DisableCodeGeneration="true">
      | 						<Type GUID="{03000018-0000-0000-E000-000000000064}">ITcWatchSource</Type>
      | 					</Interface>
      | 					<Interface>
      | 						<Type GUID="{03000010-0000-0000-E000-000000000064}">ITcCyclic</Type>
      | 					</Interface>
      | 				</Interfaces>
      | 				<Parameters>
      | 					<Parameter>
      | 						<Name>DataAreaSizes</Name>
      | 						<BitSize>64</BitSize>
      | 						<BaseType GUID="{C636B456-B483-42A5-BD8A-58753433F375}" Namespace="IO">TcIoDataAreaSize</BaseType>
      | 						<PTCID>#x0300002a</PTCID>
      | 						<ContextId>1</ContextId>
      | 					</Parameter>
      | 					<Parameter HideParameter="true">
      | 						<Name>TraceLevelMax</Name>
      | 						<Comment TxtId=""><![CDATA[Controls the amount of log messages.]]></Comment>
      | 						<BitSize>32</BitSize>
      | 						<BaseType GUID="{8007AE3B-86BB-40F2-B385-EF87FCC239A4}">TcTraceLevel</BaseType>
      | 						<PTCID>#x03002103</PTCID>
      | 						<ContextId>1</ContextId>
      | 					</Parameter>
      | 				</Parameters>
      | 				<DataAreas>
      | 					<DataArea DisableCodeGeneration="true">
      | 						<AreaNo AreaType="InputDst" CreateSymbols="true" DynamicArea="true">1</AreaNo>
      | 						<Name>Input</Name>
      | 						<ContextId>1</ContextId>
      | 						<ByteSize>4</ByteSize>
      | 						<Symbol>
      | 							<Name>MAIN.ModelToPLC</Name>
      | 							<BitSize>32</BitSize>
      | 							<BaseType GUID="{18071995-0000-0000-0000-000000000007}">DWORD</BaseType>
      | 							<PTCID>#x81000000</PTCID>
      | 							<BitOffs>0</BitOffs>
      | 						</Symbol>
      | 					</DataArea>
      | 				</DataAreas>
      | 				<InterfacePointers>
      | 					<InterfacePointer>
      | 						<PTCID>#x00000001</PTCID>
      | 						<Name>DataSink</Name>
      | 						<Type GUID="{CD026BE9-DD1E-4238-B09F-CDE426934EFB}" Namespace="TcDataExchange">ITcStreamSyncDataSink</Type>
      | 						<ContextId>1</ContextId>
      | 					</InterfacePointer>
      | 					<InterfacePointer>
      | 						<PTCID>#x03002060</PTCID>
      | 						<Name>CyclicCaller</Name>
      | 						<Type GUID="{0300001E-0000-0000-E000-000000000064}">ITcCyclicCaller</Type>
      | 						<ContextId>1</ContextId>
      | 					</InterfacePointer>
      | 				</InterfacePointers>
      | 				<InstanceName>FromDataArea_Instance1</InstanceName>
      | 				<OTCID>#x01010030</OTCID>
      | 				<ParameterValues>
      | 					<Value>
      | 						<Name>DataAreaSizes.area</Name>
      | 						<Value>1</Value>
      | 					</Value>
      | 					<Value>
      | 						<Name>DataAreaSizes.size</Name>
      | 						<Value>4</Value>
      | 					</Value>
      | 					<Value>
      | 						<Name>TraceLevelMax</Name>
      | 						<EnumText>tlAlways</EnumText>
      | 					</Value>
      | 				</ParameterValues>
      | 				<InterfacePointerValues>
      | 					<Value>
      | 						<Name>DataSink</Name>
      | 						<OTCID>#x01010020</OTCID>
      | 					</Value>
      | 					<Value>
      | 						<Name>CyclicCaller</Name>
      | 						<OTCID>#x02010020</OTCID>
      | 					</Value>
      | 				</InterfacePointerValues>
      | 			</Module>
      | 			<Module GUID="{E38BFC78-135A-4B90-A7E9-B3ECAB89AD55}" ClassFactoryId="Beckhoff Automation|TcDataExchangeModules|1.0.1.166" Group="DataExchange|Protocols">
      | 				<Name>AdsClient</Name>
      | 				<CLSID ClassFactory="TcDataExchangeModules" RealTimeInstantiable="true">{E38BFC78-135A-4B90-A7E9-B3ECAB89AD55}</CLSID>
      | 				<Info/>
      | 				<Licenses>
      | 					<License>
      | 						<LicenseId>{304D006A-8299-4560-AB79-438534B50288}</LicenseId>
      | 					</License>
      | 				</Licenses>
      | 				<InitSequence>PSO</InitSequence>
      | 				<Contexts>
      | 					<Context>
      | 						<Id>1</Id>
      | 					</Context>
      | 				</Contexts>
      | 				<Interfaces>
      | 					<Interface DisableCodeGeneration="true">
      | 						<Type GUID="{00000012-0000-0000-E000-000000000064}">ITComObject</Type>
      | 					</Interface>
      | 					<Interface DisableCodeGeneration="true">
      | 						<Type GUID="{03000012-0000-0000-E000-000000000064}">ITcADI</Type>
      | 					</Interface>
      | 					<Interface DisableCodeGeneration="true">
      | 						<Type GUID="{03000018-0000-0000-E000-000000000064}">ITcWatchSource</Type>
      | 					</Interface>
      | 					<Interface>
      | 						<Type GUID="{44CF19E6-1A23-4E07-B15E-18C86B7D1DF6}" Namespace="TcDataExchange">ITcStreamAdsClient</Type>
      | 					</Interface>
      | 				</Interfaces>
      | 				<Parameters>
      | 					<Parameter OnlineParameter="true" DisableCodeGeneration="true" ReadOnly="true">
      | 						<Name>LocalNetId</Name>
      | 						<BitSize>48</BitSize>
      | 						<BaseType GUID="{18071995-0000-0000-0000-000000000041}">AMSNETID</BaseType>
      | 						<PTCID>#x00000001</PTCID>
      | 						<ContextId>1</ContextId>
      | 					</Parameter>
      | 					<Parameter>
      | 						<Name>LocalPortNo</Name>
      | 						<BitSize>16</BitSize>
      | 						<BaseType GUID="{18071995-0000-0000-0000-000000000005}">UINT</BaseType>
      | 						<Default>
      | 							<Value>0</Value>
      | 						</Default>
      | 						<PTCID>#x00000002</PTCID>
      | 						<ContextId>1</ContextId>
      | 					</Parameter>
      | 					<Parameter>
      | 						<Name>LocalPortName</Name>
      | 						<BitSize>256</BitSize>
      | 						<BaseType GUID="{18071995-0000-0000-0000-00010000001F}">STRING(31)</BaseType>
      | 						<PTCID>#x00000003</PTCID>
      | 						<ContextId>1</ContextId>
      | 					</Parameter>
      | 					<Parameter HideParameter="true">
      | 						<Name>TraceLevelMax</Name>
      | 						<Comment TxtId=""><![CDATA[Controls the amount of log messages.]]></Comment>
      | 						<BitSize>32</BitSize>
      | 						<BaseType GUID="{8007AE3B-86BB-40F2-B385-EF87FCC239A4}">TcTraceLevel</BaseType>
      | 						<PTCID>#x03002103</PTCID>
      | 						<ContextId>1</ContextId>
      | 					</Parameter>
      | 				</Parameters>
      | 				<InstanceName>AdsClient_Instance1</InstanceName>
      | 				<OTCID>#x01010040</OTCID>
      | 				<ParameterValues>
      | 					<Value>
      | 						<Name>LocalNetId</Name>
      | 						<Data>000000000000</Data>
      | 					</Value>
      | 					<Value>
      | 						<Name>LocalPortNo</Name>
      | 						<Value>0</Value>
      | 					</Value>
      | 					<Value>
      | 						<Name>LocalPortName</Name>
      | 						<String/>
      | 					</Value>
      | 					<Value>
      | 						<Name>TraceLevelMax</Name>
      | 						<EnumText>tlAlways</EnumText>
      | 					</Value>
      | 				</ParameterValues>
      | 			</Module>
      | 			<Module GUID="{2FCAB55D-9E25-4FA5-9A83-9434B5081CA3}" ClassFactoryId="Beckhoff Automation|TcDataExchangeModules|1.0.1.166" Group="DataExchange|StreamSinkSource">
      | 				<Name>FromAndToADS</Name>
      | 				<CLSID ClassFactory="TcDataExchangeModules">{2FCAB55D-9E25-4FA5-9A83-9434B5081CA3}</CLSID>
      | 				<Info/>
      | 				<Licenses>
      | 					<License>
      | 						<LicenseId>{304D006A-8299-4560-AB79-438534B50288}</LicenseId>
      | 					</License>
      | 				</Licenses>
      | 				<InitSequence>SO</InitSequence>
      | 				<Contexts>
      | 					<Context>
      | 						<Id>1</Id>
      | 					</Context>
      | 				</Contexts>
      | 				<Interfaces>
      | 					<Interface DisableCodeGeneration="true">
      | 						<Type GUID="{00000012-0000-0000-E000-000000000064}">ITComObject</Type>
      | 					</Interface>
      | 					<Interface DisableCodeGeneration="true">
      | 						<Type GUID="{03000012-0000-0000-E000-000000000064}">ITcADI</Type>
      | 					</Interface>
      | 					<Interface DisableCodeGeneration="true">
      | 						<Type GUID="{03000018-0000-0000-E000-000000000064}">ITcWatchSource</Type>
      | 					</Interface>
      | 					<Interface>
      | 						<Type GUID="{03000010-0000-0000-E000-000000000064}">ITcCyclic</Type>
      | 					</Interface>
      | 				</Interfaces>
      | 				<Parameters>
      | 					<Parameter>
      | 						<Name>AmsAddr</Name>
      | 						<BitSize>64</BitSize>
      | 						<BaseType GUID="{18071995-0000-0000-0000-000000000042}">AMSADDR</BaseType>
      | 						<PTCID>#x00000005</PTCID>
      | 						<ContextId>1</ContextId>
      | 					</Parameter>
      | 					<Parameter>
      | 						<Name>IndexGroup</Name>
      | 						<BitSize>32</BitSize>
      | 						<BaseType GUID="{18071995-0000-0000-0000-000000000008}">UDINT</BaseType>
      | 						<PTCID>#x00000006</PTCID>
      | 						<ContextId>1</ContextId>
      | 					</Parameter>
      | 					<Parameter>
      | 						<Name>IndexOffset</Name>
      | 						<BitSize>32</BitSize>
      | 						<BaseType GUID="{18071995-0000-0000-0000-000000000008}">UDINT</BaseType>
      | 						<PTCID>#x00000007</PTCID>
      | 						<ContextId>1</ContextId>
      | 					</Parameter>
      | 					<Parameter>
      | 						<Name>ByteSize</Name>
      | 						<BitSize>32</BitSize>
      | 						<BaseType GUID="{18071995-0000-0000-0000-000000000008}">UDINT</BaseType>
      | 						<PTCID>#x00000008</PTCID>
      | 						<ContextId>1</ContextId>
      | 					</Parameter>
      | 					<Parameter>
      | 						<Name>SymbolName</Name>
      | 						<BitSize>2048</BitSize>
      | 						<BaseType GUID="{18071995-0000-0000-0000-0001000000FF}">STRING(255)</BaseType>
      | 						<PTCID>#x00000009</PTCID>
      | 						<ContextId>1</ContextId>
      | 					</Parameter>
      | 					<Parameter>
      | 						<Name>Timeout</Name>
      | 						<BitSize>32</BitSize>
      | 						<BaseType GUID="{18071995-0000-0000-0000-000000000008}">UDINT</BaseType>
      | 						<Unit><![CDATA[ms]]></Unit>
      | 						<Default>
      | 							<Value>1000</Value>
      | 						</Default>
      | 						<PTCID>#x0000000a</PTCID>
      | 						<ContextId>1</ContextId>
      | 					</Parameter>
      | 					<Parameter>
      | 						<Name>ReadViaNotification</Name>
      | 						<BitSize>8</BitSize>
      | 						<BaseType GUID="{18071995-0000-0000-0000-000000000030}">BOOL</BaseType>
      | 						<PTCID>#x0000000b</PTCID>
      | 						<ContextId>1</ContextId>
      | 					</Parameter>
      | 					<Parameter>
      | 						<Name>NotificationTransMode</Name>
      | 						<BitSize>16</BitSize>
      | 						<BaseType GUID="{2919D6B4-47C4-4AE8-B706-E94C497ECB99}" Namespace="TcDataExchange">NotificationTransMode</BaseType>
      | 						<PTCID>#x0000000c</PTCID>
      | 						<ContextId>1</ContextId>
      | 					</Parameter>
      | 					<Parameter>
      | 						<Name>NotificationSampleTime</Name>
      | 						<BitSize>32</BitSize>
      | 						<BaseType GUID="{18071995-0000-0000-0000-000000000008}">UDINT</BaseType>
      | 						<PTCID>#x0000000d</PTCID>
      | 						<ContextId>1</ContextId>
      | 					</Parameter>
      | 					<Parameter>
      | 						<Name>NotificationDelayTime</Name>
      | 						<BitSize>32</BitSize>
      | 						<BaseType GUID="{18071995-0000-0000-0000-000000000008}">UDINT</BaseType>
      | 						<PTCID>#x0000000e</PTCID>
      | 						<ContextId>1</ContextId>
      | 					</Parameter>
      | 					<Parameter HideParameter="true">
      | 						<Name>TraceLevelMax</Name>
      | 						<Comment TxtId=""><![CDATA[Controls the amount of log messages.]]></Comment>
      | 						<BitSize>32</BitSize>
      | 						<BaseType GUID="{8007AE3B-86BB-40F2-B385-EF87FCC239A4}">TcTraceLevel</BaseType>
      | 						<PTCID>#x03002103</PTCID>
      | 						<ContextId>1</ContextId>
      | 					</Parameter>
      | 				</Parameters>
      | 				<InterfacePointers>
      | 					<InterfacePointer>
      | 						<PTCID>#x00000001</PTCID>
      | 						<Name>AdsClient</Name>
      | 						<Type GUID="{44CF19E6-1A23-4E07-B15E-18C86B7D1DF6}" Namespace="TcDataExchange">ITcStreamAdsClient</Type>
      | 						<ContextId>1</ContextId>
      | 					</InterfacePointer>
      | 					<InterfacePointer>
      | 						<PTCID>#x03002060</PTCID>
      | 						<Name>CyclicCaller</Name>
      | 						<Type GUID="{0300001E-0000-0000-E000-000000000064}">ITcCyclicCaller</Type>
      | 						<ContextId>1</ContextId>
      | 					</InterfacePointer>
      | 					<InterfacePointer>
      | 						<PTCID>#x00000003</PTCID>
      | 						<Name>DataSource</Name>
      | 						<Type GUID="{877CB26F-4EC1-469B-9F87-706DDBDA821F}" Namespace="TcDataExchange">ITcStreamSyncDataSource</Type>
      | 						<ContextId>1</ContextId>
      | 					</InterfacePointer>
      | 					<InterfacePointer>
      | 						<PTCID>#x00000004</PTCID>
      | 						<Name>DataSink</Name>
      | 						<Type GUID="{CD026BE9-DD1E-4238-B09F-CDE426934EFB}" Namespace="TcDataExchange">ITcStreamSyncDataSink</Type>
      | 						<ContextId>1</ContextId>
      | 					</InterfacePointer>
      | 				</InterfacePointers>
      | 				<InstanceName>FromAndToADS_Instance1</InstanceName>
      | 				<OTCID>#x01010050</OTCID>
      | 				<ParameterValues>
      | 					<Value>
      | 						<Name>AmsAddr.netId</Name>
      | 						<Data>c0a8089b0101</Data>
      | 					</Value>
      | 					<Value>
      | 						<Name>AmsAddr.port</Name>
      | 						<Value>851</Value>
      | 					</Value>
      | 					<Value>
      | 						<Name>IndexGroup</Name>
      | 						<Value>0</Value>
      | 					</Value>
      | 					<Value>
      | 						<Name>IndexOffset</Name>
      | 						<Value>0</Value>
      | 					</Value>
      | 					<Value>
      | 						<Name>ByteSize</Name>
      | 						<Value>4</Value>
      | 					</Value>
      | 					<Value>
      | 						<Name>SymbolName</Name>
      | 						<String>MAIN.ModelToPLC</String>
      | 					</Value>
      | 					<Value>
      | 						<Name>Timeout</Name>
      | 						<Value>1000</Value>
      | 					</Value>
      | 					<Value>
      | 						<Name>ReadViaNotification</Name>
      | 						<EnumText>FALSE</EnumText>
      | 					</Value>
      | 					<Value>
      | 						<Name>NotificationTransMode</Name>
      | 						<EnumText>NoTrans</EnumText>
      | 					</Value>
      | 					<Value>
      | 						<Name>NotificationSampleTime</Name>
      | 						<Value>0</Value>
      | 					</Value>
      | 					<Value>
      | 						<Name>NotificationDelayTime</Name>
      | 						<Value>0</Value>
      | 					</Value>
      | 					<Value>
      | 						<Name>TraceLevelMax</Name>
      | 						<EnumText>tlAlways</EnumText>
      | 					</Value>
      | 				</ParameterValues>
      | 				<InterfacePointerValues>
      | 					<Value>
      | 						<Name>AdsClient</Name>
      | 						<OTCID>#x01010040</OTCID>
      | 					</Value>
      | 					<Value>
      | 						<Name>CyclicCaller</Name>
      | 						<OTCID>#x02010020</OTCID>
      | 					</Value>
      | 					<Value>
      | 						<Name>DataSource</Name>
      | 						<OTCID>#x01010020</OTCID>
      | 					</Value>
      | 					<Value>
      | 						<Name>DataSink</Name>
      | 						<OTCID>#x00000000</OTCID>
      | 					</Value>
      | 				</InterfacePointerValues>
      | 			</Module>
      | 			<Module GUID="{7F2917A9-6092-40A6-BB22-5428D680BA27}" ClassFactoryId="Beckhoff Automation|TcDataExchangeModules|1.0.1.166" Group="DataExchange|StreamUtilities">
      | 				<Name>SyncBuffer</Name>
      | 				<CLSID ClassFactory="TcDataExchangeModules">{7F2917A9-6092-40A6-BB22-5428D680BA27}</CLSID>
      | 				<Info/>
      | 				<Licenses>
      | 					<License>
      | 						<LicenseId>{304D006A-8299-4560-AB79-438534B50288}</LicenseId>
      | 					</License>
      | 				</Licenses>
      | 				<InitSequence>SO</InitSequence>
      | 				<Contexts>
      | 					<Context>
      | 						<Id>1</Id>
      | 					</Context>
      | 				</Contexts>
      | 				<Interfaces>
      | 					<Interface DisableCodeGeneration="true">
      | 						<Type GUID="{00000012-0000-0000-E000-000000000064}">ITComObject</Type>
      | 					</Interface>
      | 					<Interface DisableCodeGeneration="true">
      | 						<Type GUID="{03000012-0000-0000-E000-000000000064}">ITcADI</Type>
      | 					</Interface>
      | 					<Interface DisableCodeGeneration="true">
      | 						<Type GUID="{03000018-0000-0000-E000-000000000064}">ITcWatchSource</Type>
      | 					</Interface>
      | 					<Interface>
      | 						<Type GUID="{CD026BE9-DD1E-4238-B09F-CDE426934EFB}" Namespace="TcDataExchange">ITcStreamSyncDataSink</Type>
      | 					</Interface>
      | 					<Interface>
      | 						<Type GUID="{877CB26F-4EC1-469B-9F87-706DDBDA821F}" Namespace="TcDataExchange">ITcStreamSyncDataSource</Type>
      | 					</Interface>
      | 					<Interface>
      | 						<Type GUID="{CC2323D2-5F91-43AC-9820-54D42A9D0317}" Namespace="TcDataExchange">ITcStreamBuffer</Type>
      | 					</Interface>
      | 				</Interfaces>
      | 				<Parameters>
      | 					<Parameter>
      | 						<Name>InterpolationMode</Name>
      | 						<BitSize>16</BitSize>
      | 						<BaseType GUID="{04A85163-BBE2-45EF-A167-1FD20C2F2D46}" Namespace="TcDataExchange">BufferReadInterpolationMode</BaseType>
      | 						<PTCID>#x00000004</PTCID>
      | 						<ContextId>1</ContextId>
      | 					</Parameter>
      | 					<Parameter>
      | 						<Name>ContinuationMode</Name>
      | 						<BitSize>16</BitSize>
      | 						<BaseType GUID="{B2873DF7-0E9A-4371-8FDA-560A407550FC}" Namespace="TcDataExchange">BufferReadExtrapolationMode</BaseType>
      | 						<PTCID>#x00000005</PTCID>
      | 						<ContextId>1</ContextId>
      | 					</Parameter>
      | 					<Parameter>
      | 						<Name>SampleSize</Name>
      | 						<BitSize>32</BitSize>
      | 						<BaseType GUID="{18071995-0000-0000-0000-000000000008}">UDINT</BaseType>
      | 						<PTCID>#x00000006</PTCID>
      | 						<ContextId>1</ContextId>
      | 					</Parameter>
      | 					<Parameter>
      | 						<Name>Capacity</Name>
      | 						<BitSize>32</BitSize>
      | 						<BaseType GUID="{18071995-0000-0000-0000-000000000008}">UDINT</BaseType>
      | 						<PTCID>#x00000007</PTCID>
      | 						<ContextId>1</ContextId>
      | 					</Parameter>
      | 					<Parameter HideParameter="true">
      | 						<Name>TraceLevelMax</Name>
      | 						<Comment TxtId=""><![CDATA[Controls the amount of log messages.]]></Comment>
      | 						<BitSize>32</BitSize>
      | 						<BaseType GUID="{8007AE3B-86BB-40F2-B385-EF87FCC239A4}">TcTraceLevel</BaseType>
      | 						<PTCID>#x03002103</PTCID>
      | 						<ContextId>1</ContextId>
      | 					</Parameter>
      | 				</Parameters>
      | 				<InterfacePointers>
      | 					<InterfacePointer>
      | 						<PTCID>#x00000001</PTCID>
      | 						<Name>Synchronizer</Name>
      | 						<Type GUID="{9165C8A1-78D1-4B81-89D0-BA48F61AF93B}" Namespace="TcDataExchange">ITcStreamSynchronizer</Type>
      | 						<ContextId>1</ContextId>
      | 					</InterfacePointer>
      | 				</InterfacePointers>
      | 				<InstanceName>SyncBuffer_Instance2</InstanceName>
      | 				<OTCID>#x01010060</OTCID>
      | 				<ParameterValues>
      | 					<Value>
      | 						<Name>InterpolationMode</Name>
      | 						<EnumText>InterpolationMode_Nearest</EnumText>
      | 					</Value>
      | 					<Value>
      | 						<Name>ContinuationMode</Name>
      | 						<EnumText>ExtrapolationMode_None</EnumText>
      | 					</Value>
      | 					<Value>
      | 						<Name>SampleSize</Name>
      | 						<Value>4</Value>
      | 					</Value>
      | 					<Value>
      | 						<Name>Capacity</Name>
      | 						<Value>50</Value>
      | 					</Value>
      | 					<Value>
      | 						<Name>TraceLevelMax</Name>
      | 						<EnumText>tlAlways</EnumText>
      | 					</Value>
      | 				</ParameterValues>
      | 				<InterfacePointerValues>
      | 					<Value>
      | 						<Name>Synchronizer</Name>
      | 						<OTCID>#x01010010</OTCID>
      | 					</Value>
      | 				</InterfacePointerValues>
      | 			</Module>
      | 			<Module GUID="{2FCAB55D-9E25-4FA5-9A83-9434B5081CA3}" ClassFactoryId="Beckhoff Automation|TcDataExchangeModules|1.0.1.166" Group="DataExchange|StreamSinkSource">
      | 				<Name>FromAndToADS</Name>
      | 				<CLSID ClassFactory="TcDataExchangeModules">{2FCAB55D-9E25-4FA5-9A83-9434B5081CA3}</CLSID>
      | 				<Info/>
      | 				<Licenses>
      | 					<License>
      | 						<LicenseId>{304D006A-8299-4560-AB79-438534B50288}</LicenseId>
      | 					</License>
      | 				</Licenses>
      | 				<InitSequence>SO</InitSequence>
      | 				<Contexts>
      | 					<Context>
      | 						<Id>1</Id>
      | 					</Context>
      | 				</Contexts>
      | 				<Interfaces>
      | 					<Interface DisableCodeGeneration="true">
      | 						<Type GUID="{00000012-0000-0000-E000-000000000064}">ITComObject</Type>
      | 					</Interface>
      | 					<Interface DisableCodeGeneration="true">
      | 						<Type GUID="{03000012-0000-0000-E000-000000000064}">ITcADI</Type>
      | 					</Interface>
      | 					<Interface DisableCodeGeneration="true">
      | 						<Type GUID="{03000018-0000-0000-E000-000000000064}">ITcWatchSource</Type>
      | 					</Interface>
      | 					<Interface>
      | 						<Type GUID="{03000010-0000-0000-E000-000000000064}">ITcCyclic</Type>
      | 					</Interface>
      | 				</Interfaces>
      | 				<Parameters>
      | 					<Parameter>
      | 						<Name>AmsAddr</Name>
      | 						<BitSize>64</BitSize>
      | 						<BaseType GUID="{18071995-0000-0000-0000-000000000042}">AMSADDR</BaseType>
      | 						<PTCID>#x00000005</PTCID>
      | 						<ContextId>1</ContextId>
      | 					</Parameter>
      | 					<Parameter>
      | 						<Name>IndexGroup</Name>
      | 						<BitSize>32</BitSize>
      | 						<BaseType GUID="{18071995-0000-0000-0000-000000000008}">UDINT</BaseType>
      | 						<PTCID>#x00000006</PTCID>
      | 						<ContextId>1</ContextId>
      | 					</Parameter>
      | 					<Parameter>
      | 						<Name>IndexOffset</Name>
      | 						<BitSize>32</BitSize>
      | 						<BaseType GUID="{18071995-0000-0000-0000-000000000008}">UDINT</BaseType>
      | 						<PTCID>#x00000007</PTCID>
      | 						<ContextId>1</ContextId>
      | 					</Parameter>
      | 					<Parameter>
      | 						<Name>ByteSize</Name>
      | 						<BitSize>32</BitSize>
      | 						<BaseType GUID="{18071995-0000-0000-0000-000000000008}">UDINT</BaseType>
      | 						<PTCID>#x00000008</PTCID>
      | 						<ContextId>1</ContextId>
      | 					</Parameter>
      | 					<Parameter>
      | 						<Name>SymbolName</Name>
      | 						<BitSize>2048</BitSize>
      | 						<BaseType GUID="{18071995-0000-0000-0000-0001000000FF}">STRING(255)</BaseType>
      | 						<PTCID>#x00000009</PTCID>
      | 						<ContextId>1</ContextId>
      | 					</Parameter>
      | 					<Parameter>
      | 						<Name>Timeout</Name>
      | 						<BitSize>32</BitSize>
      | 						<BaseType GUID="{18071995-0000-0000-0000-000000000008}">UDINT</BaseType>
      | 						<Unit><![CDATA[ms]]></Unit>
      | 						<Default>
      | 							<Value>1000</Value>
      | 						</Default>
      | 						<PTCID>#x0000000a</PTCID>
      | 						<ContextId>1</ContextId>
      | 					</Parameter>
      | 					<Parameter>
      | 						<Name>ReadViaNotification</Name>
      | 						<BitSize>8</BitSize>
      | 						<BaseType GUID="{18071995-0000-0000-0000-000000000030}">BOOL</BaseType>
      | 						<PTCID>#x0000000b</PTCID>
      | 						<ContextId>1</ContextId>
      | 					</Parameter>
      | 					<Parameter>
      | 						<Name>NotificationTransMode</Name>
      | 						<BitSize>16</BitSize>
      | 						<BaseType GUID="{2919D6B4-47C4-4AE8-B706-E94C497ECB99}" Namespace="TcDataExchange">NotificationTransMode</BaseType>
      | 						<PTCID>#x0000000c</PTCID>
      | 						<ContextId>1</ContextId>
      | 					</Parameter>
      | 					<Parameter>
      | 						<Name>NotificationSampleTime</Name>
      | 						<BitSize>32</BitSize>
      | 						<BaseType GUID="{18071995-0000-0000-0000-000000000008}">UDINT</BaseType>
      | 						<PTCID>#x0000000d</PTCID>
      | 						<ContextId>1</ContextId>
      | 					</Parameter>
      | 					<Parameter>
      | 						<Name>NotificationDelayTime</Name>
      | 						<BitSize>32</BitSize>
      | 						<BaseType GUID="{18071995-0000-0000-0000-000000000008}">UDINT</BaseType>
      | 						<PTCID>#x0000000e</PTCID>
      | 						<ContextId>1</ContextId>
      | 					</Parameter>
      | 					<Parameter HideParameter="true">
      | 						<Name>TraceLevelMax</Name>
      | 						<Comment TxtId=""><![CDATA[Controls the amount of log messages.]]></Comment>
      | 						<BitSize>32</BitSize>
      | 						<BaseType GUID="{8007AE3B-86BB-40F2-B385-EF87FCC239A4}">TcTraceLevel</BaseType>
      | 						<PTCID>#x03002103</PTCID>
      | 						<ContextId>1</ContextId>
      | 					</Parameter>
      | 				</Parameters>
      | 				<InterfacePointers>
      | 					<InterfacePointer>
      | 						<PTCID>#x00000001</PTCID>
      | 						<Name>AdsClient</Name>
      | 						<Type GUID="{44CF19E6-1A23-4E07-B15E-18C86B7D1DF6}" Namespace="TcDataExchange">ITcStreamAdsClient</Type>
      | 						<ContextId>1</ContextId>
      | 					</InterfacePointer>
      | 					<InterfacePointer>
      | 						<PTCID>#x03002060</PTCID>
      | 						<Name>CyclicCaller</Name>
      | 						<Type GUID="{0300001E-0000-0000-E000-000000000064}">ITcCyclicCaller</Type>
      | 						<ContextId>1</ContextId>
      | 					</InterfacePointer>
      | 					<InterfacePointer>
      | 						<PTCID>#x00000003</PTCID>
      | 						<Name>DataSource</Name>
      | 						<Type GUID="{877CB26F-4EC1-469B-9F87-706DDBDA821F}" Namespace="TcDataExchange">ITcStreamSyncDataSource</Type>
      | 						<ContextId>1</ContextId>
      | 					</InterfacePointer>
      | 					<InterfacePointer>
      | 						<PTCID>#x00000004</PTCID>
      | 						<Name>DataSink</Name>
      | 						<Type GUID="{CD026BE9-DD1E-4238-B09F-CDE426934EFB}" Namespace="TcDataExchange">ITcStreamSyncDataSink</Type>
      | 						<ContextId>1</ContextId>
      | 					</InterfacePointer>
      | 				</InterfacePointers>
      | 				<InstanceName>FromAndToADS_Instance2</InstanceName>
      | 				<OTCID>#x01010070</OTCID>
      | 				<ParameterValues>
      | 					<Value>
      | 						<Name>AmsAddr.netId</Name>
      | 						<Data>c0a8089b0101</Data>
      | 					</Value>
      | 					<Value>
      | 						<Name>AmsAddr.port</Name>
      | 						<Value>851</Value>
      | 					</Value>
      | 					<Value>
      | 						<Name>IndexGroup</Name>
      | 						<Value>0</Value>
      | 					</Value>
      | 					<Value>
      | 						<Name>IndexOffset</Name>
      | 						<Value>0</Value>
      | 					</Value>
      | 					<Value>
      | 						<Name>ByteSize</Name>
      | 						<Value>4</Value>
      | 					</Value>
      | 					<Value>
      | 						<Name>SymbolName</Name>
      | 						<String>MAIN.PLCToModel</String>
      | 					</Value>
      | 					<Value>
      | 						<Name>Timeout</Name>
      | 						<Value>1000</Value>
      | 					</Value>
      | 					<Value>
      | 						<Name>ReadViaNotification</Name>
      | 						<EnumText>TRUE</EnumText>
      | 					</Value>
      | 					<Value>
      | 						<Name>NotificationTransMode</Name>
      | 						<EnumText>ServerCycle</EnumText>
      | 					</Value>
      | 					<Value>
      | 						<Name>NotificationSampleTime</Name>
      | 						<Value>100000</Value>
      | 					</Value>
      | 					<Value>
      | 						<Name>NotificationDelayTime</Name>
      | 						<Value>1000000</Value>
      | 					</Value>
      | 					<Value>
      | 						<Name>TraceLevelMax</Name>
      | 						<EnumText>tlAlways</EnumText>
      | 					</Value>
      | 				</ParameterValues>
      | 				<InterfacePointerValues>
      | 					<Value>
      | 						<Name>AdsClient</Name>
      | 						<OTCID>#x01010040</OTCID>
      | 					</Value>
      | 					<Value>
      | 						<Name>CyclicCaller</Name>
      | 						<OTCID>#x02010020</OTCID>
      | 					</Value>
      | 					<Value>
      | 						<Name>DataSource</Name>
      | 						<OTCID>#x00000000</OTCID>
      | 					</Value>
      | 					<Value>
      | 						<Name>DataSink</Name>
      | 						<OTCID>#x01010060</OTCID>
      | 					</Value>
      | 				</InterfacePointerValues>
      | 			</Module>
      | 			<Module GUID="{0D48E1A1-2F46-4184-A85B-04744F5D3239}" ClassFactoryId="Beckhoff Automation|TcDataExchangeModules|1.0.1.166" Group="DataExchange|StreamSinkSource">
      | 				<Name>ToDataArea</Name>
      | 				<CLSID ClassFactory="TcDataExchangeModules">{0D48E1A1-2F46-4184-A85B-04744F5D3239}</CLSID>
      | 				<Info/>
      | 				<Licenses>
      | 					<License>
      | 						<LicenseId>{304D006A-8299-4560-AB79-438534B50288}</LicenseId>
      | 					</License>
      | 				</Licenses>
      | 				<InitSequence>SO</InitSequence>
      | 				<Contexts>
      | 					<Context>
      | 						<Id>1</Id>
      | 					</Context>
      | 				</Contexts>
      | 				<Interfaces>
      | 					<Interface DisableCodeGeneration="true">
      | 						<Type GUID="{00000012-0000-0000-E000-000000000064}">ITComObject</Type>
      | 					</Interface>
      | 					<Interface DisableCodeGeneration="true">
      | 						<Type GUID="{03000012-0000-0000-E000-000000000064}">ITcADI</Type>
      | 					</Interface>
      | 					<Interface DisableCodeGeneration="true">
      | 						<Type GUID="{03000018-0000-0000-E000-000000000064}">ITcWatchSource</Type>
      | 					</Interface>
      | 					<Interface>
      | 						<Type GUID="{03000010-0000-0000-E000-000000000064}">ITcCyclic</Type>
      | 					</Interface>
      | 				</Interfaces>
      | 				<Parameters>
      | 					<Parameter>
      | 						<Name>DataAreaSizes</Name>
      | 						<BitSize>64</BitSize>
      | 						<BaseType GUID="{C636B456-B483-42A5-BD8A-58753433F375}" Namespace="IO">TcIoDataAreaSize</BaseType>
      | 						<PTCID>#x0300002a</PTCID>
      | 						<ContextId>1</ContextId>
      | 					</Parameter>
      | 					<Parameter HideParameter="true">
      | 						<Name>TraceLevelMax</Name>
      | 						<Comment TxtId=""><![CDATA[Controls the amount of log messages.]]></Comment>
      | 						<BitSize>32</BitSize>
      | 						<BaseType GUID="{8007AE3B-86BB-40F2-B385-EF87FCC239A4}">TcTraceLevel</BaseType>
      | 						<PTCID>#x03002103</PTCID>
      | 						<ContextId>1</ContextId>
      | 					</Parameter>
      | 				</Parameters>
      | 				<DataAreas>
      | 					<DataArea DisableCodeGeneration="true">
      | 						<AreaNo AreaType="OutputSrc" CreateSymbols="true" DynamicArea="true">1</AreaNo>
      | 						<Name>Output</Name>
      | 						<ContextId>1</ContextId>
      | 						<ByteSize>4</ByteSize>
      | 						<Symbol>
      | 							<Name>MAIN.PLCToModel</Name>
      | 							<BitSize>32</BitSize>
      | 							<BaseType GUID="{18071995-0000-0000-0000-000000000007}">DWORD</BaseType>
      | 							<PTCID>#x81000000</PTCID>
      | 							<BitOffs>0</BitOffs>
      | 						</Symbol>
      | 					</DataArea>
      | 				</DataAreas>
      | 				<InterfacePointers>
      | 					<InterfacePointer>
      | 						<PTCID>#x00000001</PTCID>
      | 						<Name>DataSource</Name>
      | 						<Type GUID="{877CB26F-4EC1-469B-9F87-706DDBDA821F}" Namespace="TcDataExchange">ITcStreamSyncDataSource</Type>
      | 						<ContextId>1</ContextId>
      | 					</InterfacePointer>
      | 					<InterfacePointer>
      | 						<PTCID>#x03002060</PTCID>
      | 						<Name>CyclicCaller</Name>
      | 						<Type GUID="{0300001E-0000-0000-E000-000000000064}">ITcCyclicCaller</Type>
      | 						<ContextId>1</ContextId>
      | 					</InterfacePointer>
      | 				</InterfacePointers>
      | 				<InstanceName>ToDataArea_Instance1</InstanceName>
      | 				<OTCID>#x01010080</OTCID>
      | 				<ParameterValues>
      | 					<Value>
      | 						<Name>DataAreaSizes.area</Name>
      | 						<Value>1</Value>
      | 					</Value>
      | 					<Value>
      | 						<Name>DataAreaSizes.size</Name>
      | 						<Value>4</Value>
      | 					</Value>
      | 					<Value>
      | 						<Name>TraceLevelMax</Name>
      | 						<EnumText>tlAlways</EnumText>
      | 					</Value>
      | 				</ParameterValues>
      | 				<InterfacePointerValues>
      | 					<Value>
      | 						<Name>DataSource</Name>
      | 						<OTCID>#x01010060</OTCID>
      | 					</Value>
      | 					<Value>
      | 						<Name>CyclicCaller</Name>
      | 						<OTCID>#x02010020</OTCID>
      | 					</Value>
      | 				</InterfacePointerValues>
      | 			</Module>
      | 		</Modules>
      | 	</System>
      | </TcRuntimAdapterProject>
      SymbolInterfaceInfo=|
      | <PortInfo>
      | 	<Inputs>
      | 		<SymbolControlItems>
      | 			<SymbolControlItem GroupName="ADS Write" GroupDescription="Parameters for ADS Write command">
      | 				<Parameters>
      | 					<Parameter Name="Name">MAIN.ModelToPLC</Parameter>
      | 					<Parameter Name="SymbolName">MAIN.ModelToPLC</Parameter>
      | 					<Parameter Name="SymbolType">DWORD</Parameter>
      | 					<Parameter Name="SymbolGuid">{18071995-0000-0000-0000-000000000007}</Parameter>
      | 					<Parameter Name="AmsNetId">192.168.8.155.1.1</Parameter>
      | 					<Parameter Name="Port">851</Parameter>
      | 					<Parameter Name="IndexGroup">#x0</Parameter>
      | 					<Parameter Name="IndexOffset">#x0</Parameter>
      | 					<Parameter Name="BitSize">32</Parameter>
      | 					<Parameter Name="InterpolationMode">3</Parameter>
      | 					<Parameter Name="ExtrapolationMode">0</Parameter>
      | 					<Parameter Name="SampleTime TC[100ns]">100000</Parameter>
      | 					<Parameter Name="SampleTime">100000</Parameter>
      | 					<Parameter Name="Timeout">1000</Parameter>
      | 					<Parameter Name="BufferSize">50</Parameter>
      | 				</Parameters>
      | 			</SymbolControlItem>
      | 		</SymbolControlItems>
      | 	</Inputs>
      | 	<Outputs>
      | 		<SymbolControlItems>
      | 			<SymbolControlItem GroupName="ADS Read" GroupDescription="Parameters for ADS Read command">
      | 				<Parameters>
      | 					<Parameter Name="Name">MAIN.PLCToModel</Parameter>
      | 					<Parameter Name="SymbolName">MAIN.PLCToModel</Parameter>
      | 					<Parameter Name="SymbolType">DWORD</Parameter>
      | 					<Parameter Name="SymbolGuid">{18071995-0000-0000-0000-000000000007}</Parameter>
      | 					<Parameter Name="AmsNetId">192.168.8.155.1.1</Parameter>
      | 					<Parameter Name="Port">851</Parameter>
      | 					<Parameter Name="IndexGroup">#x0</Parameter>
      | 					<Parameter Name="IndexOffset">#x0</Parameter>
      | 					<Parameter Name="BitSize">32</Parameter>
      | 					<Parameter Name="InterpolationMode">3</Parameter>
      | 					<Parameter Name="ExtrapolationMode">0</Parameter>
      | 					<Parameter Name="SampleTime TC[100ns]">100000</Parameter>
      | 					<Parameter Name="SampleTime">100000</Parameter>
      | 					<Parameter Name="ReadViaNotification">True</Parameter>
      | 					<Parameter Name="Transmode">3</Parameter>
      | 					<Parameter Name="Timeout">1000</Parameter>
      | 					<Parameter Name="DelayTime">1000000</Parameter>
      | 					<Parameter Name="BufferSize">50</Parameter>
      | 				</Parameters>
      | 			</SymbolControlItem>
      | 		</SymbolControlItems>
      | 	</Outputs>
      | </PortInfo>
      settings: SourceProductName=Beckhoff TwinCAT Interface
  Scope : Scope  NumInputPorts=2
  Step : Step  Time=0.5  SampleTime=0
  wires:
  Encode/1(modelToPlc) -> PLC Communictaion/1  "MAIN.ModelToPLC"
  Cast/1 -> Encode/2(driveState)
  PLC Communictaion/1 -> Cast3/1  "MAIN.PLCToModel"
  Cast3/1 -> Decode/1(PlcToModel)
  Data Type Conversion/1 -> Encode/1(counterValue)
  Constant3/1 -> Model1/1
  Model1/2 -> Cast/1
  Model1/1 -> Data Type Conversion/1
  Model1/8 -> Scope/2
  Model1/6 -> Display1/1
  Model1/5 -> Display2/1
  Model1/4 -> Display3/1
  Model1/3 -> Display6/1
  Constant6/1 -> Model1/4
  Model1/7 -> Scope/1
  Step/1 -> Cast To Boolean/1
  Cast To Boolean/1 -> Model1/2
